simulink model "ROM_draft2"  (R2023a)
settings: Solver=ode15s  StartTime=0.0  StopTime=3  FixedStep=0.1  RelTol=1e-3
model workspace (MAT data in the model file):
  E_IVD4_N = 5
  E_IVD4_Z1 = 5
  E_IVD4_Z2 = 5
  E_IVD4_Z3 = 5
  E_IVD4_Z4 = 5
  E_IVD5_N = 5
  E_IVD5_Z1 = 5
  E_IVD5_Z2 = 5
  E_IVD5_Z3 = 5
  E_IVD5_Z4 = 5
  IVD5_N.InterfaceFrameOrigins = [0.00119634453319  0.0658349886468  0.905560470856; 0.000738781111538  0.0718151805359  0.915203379453]
  IVD5_N.InterfaceFrameOrientations = [0.963982062514  -0.265850048581  -0.0076111073418  0.00209901546435; 0.970389572461  -0.241521069818  0.00331223233616  -0.000824384267944]
  IVD5_N.StiffnessMatrix = [12072.1210467 -274.061579069 -476.370544654 -0.0848536559846 34.5351827952 -19.5673133357 -12072.1210467 274.061579068 476.370544653 -0.121182854467 81.6572072926 -52.5008864779 ... (196 elements, 14x14)]
  IVD5_N.MassMatrix = [0.00145261006911 -3.28751977521e-05 -5.02520057009e-05 2.70896299944e-09 3.95047279511e-07 -1.70980551184e-07 0.000938457476927 1.77908731253e-05 3.15075839837e-05 -9.24765904888e-09 -2.48315227579e-06 1.67944140759e-06 ... (196 elements, 14x14)]
  IVD5_N.GraphicVertexCoordinates = [-0.0121724567413 -0.0105574836731 -0.0114222154617 -0.0129605951309 -0.0126794233322 -0.0115785064697 -0.0118535032272 -0.00319156455994 -0.00319188046455 -0.00571438598633 -4.47452294499e-05 0.00311250649847 ... (1698 elements, 566x3)]
  IVD5_N.GraphicFacetVertexIndices = [1 4 5 8 11 14 17 20 23 26 28 31 ... (3384 elements, 1128x3)]
  IVD5_N.GraphicReconstructionMatrix = [0.339186715765 -0.0243256844818 -0.186223853856 0.294199181327 -0.00640190377512 -0.15234196868 0.195526379715 -0.0060796942636 -0.142913155438 0.244126675106 -0.0106723088514 -0.158139775185 ... (23772 elements, 1698x14)]
  IVD5_Z1.InterfaceFrameOrigins = [0.000873550632761  0.0769295550328  0.898954504373; 0.00103448042212  0.0848390231016  0.908281981027]
  IVD5_Z1.InterfaceFrameOrientations = [0.963982062514  -0.265850048581  -0.0076111073418  0.00209901546435; 0.970389572461  -0.241521069818  0.00331223233616  -0.000824384267944]
  IVD5_Z1.StiffnessMatrix = [5996.43220354 4.30460635168 53.0071518463 0.68427648579 19.4752112689 -31.152810894 -5996.43220354 -4.3046063519 -53.0071518468 -0.305169226095 36.4478396857 -16.2750854071 ... (196 elements, 14x14)]
  IVD5_Z1.MassMatrix = [0.00101136411122 -1.06281560629e-05 -1.3336781227e-05 -3.7152952177e-08 9.78126965242e-08 -1.12543471379e-06 0.00055045795202 6.98371650339e-06 1.00424226413e-05 1.09339655695e-08 -1.9997764811e-06 4.03451089866e-07 ... (196 elements, 14x14)]
  IVD5_Z1.GraphicVertexCoordinates = [-0.00849552154541 -0.00710174512863 -0.00716232396796 -0.0142471482979 -0.0153294525146 -0.0152496709824 -0.00567360639572 -0.00564802122116 -0.00557869402219 -0.00564833688736 -0.00567392206192 0.00247848033905 ... (1554 elements, 518x3)]
  IVD5_Z1.GraphicFacetVertexIndices = [1 4 7 10 10 12 15 18 20 23 26 29 ... (3096 elements, 1032x3)]
  IVD5_Z1.GraphicReconstructionMatrix = [0.199445115194 -0.0696803209522 -0.0744700855901 0.0059035639951 -0.000379739053346 -0.0013061688012 0.0307297998401 -0.0137062851462 -0.0106957383637 0.40254283486 -0.169685115848 -0.185804981554 ... (21756 elements, 1554x14)]
  IVD5_Z2.InterfaceFrameOrigins = [0.000604761990392  0.0571888576031  0.910711195808; 4.49988118865e-05  0.0600241328211  0.921467825643]
  IVD5_Z2.InterfaceFrameOrientations = [0.963982062514  -0.265850048581  -0.0076111073418  0.00209901546435; 0.970389572461  -0.241521069818  0.00331223233616  -0.000824384267944]
  IVD5_Z2.StiffnessMatrix = [3182.87404983 7.23028304405 -81.8198650663 -0.0684213777452 14.0226472063 0.101851145356 -3182.87404983 -7.23028304422 81.8198650673 -0.241333936335 20.1685510133 -9.13022230709 ... (196 elements, 14x14)]
  IVD5_Z2.MassMatrix = [0.000320666483951 4.44068362481e-07 -1.92499536011e-07 -4.69532859899e-09 2.63976402041e-07 3.85211947716e-08 0.000231555416641 1.63281867833e-06 7.22837907777e-07 7.7167688392e-09 -8.23428240926e-07 4.59263039163e-07 ... (196 elements, 14x14)]
  IVD5_Z2.GraphicVertexCoordinates = [0.0116057628963 0.0122282781601 0.0116208400726 -0.0131143016815 -0.0129614706039 -0.0126898040771 -0.0121298876402 -0.0133299627304 -0.0129422960281 -0.0121591796875 -0.0137408895493 -0.0137489080429 ... (1266 elements, 422x3)]
  IVD5_Z2.GraphicFacetVertexIndices = [1 4 4 4 4 9 12 14 17 20 23 25 ... (2520 elements, 840x3)]
  IVD5_Z2.GraphicReconstructionMatrix = [0.022905241299 -0.0160356716758 0.0172326687077 0.174782421627 -0.0165100138029 0.159517344737 0.0018288444813 -0.00446676244893 0.00273822898953 0.452008736901 0.0398453014282 -0.281808352519 ... (17724 elements, 1266x14)]
  IVD5_Z3.InterfaceFrameOrigins = [-0.0141350531982  0.0665747464449  0.90484779108; -0.0154737618286  0.0716573347521  0.915406801231]
  IVD5_Z3.InterfaceFrameOrientations = [0.963982062514  -0.265850048581  -0.0076111073418  0.00209901546435; 0.970389572461  -0.241521069818  0.00331223233616  -0.000824384267944]
  IVD5_Z3.StiffnessMatrix = [4692.3946555 -372.737703142 -764.852122067 4.59128038682 24.6626166315 -13.5635629732 -4692.3946555 372.737703142 764.852122068 -4.54296764783 23.8605120342 -9.7869600556 ... (196 elements, 14x14)]
  IVD5_Z3.MassMatrix = [0.00108979588426 -7.91948772423e-05 -0.00012971252151 -3.95532003515e-07 6.16575573035e-07 -1.62927188642e-06 0.000430209135056 4.56023636695e-05 7.63206897759e-05 3.12965499465e-07 -1.54222628864e-06 5.60394961299e-08 ... (196 elements, 14x14)]
  IVD5_Z3.GraphicVertexCoordinates = [-0.0119716072083 -0.0115785064697 -0.010625453949 -0.0105742545404 -0.00962718868256 -0.0102103004456 -0.00961538410187 -0.00823415184021 -0.00846083084375 -0.00981032980596 -0.0216970863342 -0.0212184925079 ... (1647 elements, 549x3)]
  IVD5_Z3.GraphicFacetVertexIndices = [1 4 7 5 11 11 16 19 22 25 28 28 ... (3282 elements, 1094x3)]
  IVD5_Z3.GraphicReconstructionMatrix = [0.840714753705 0.0133701682388 0.0301596742866 0.935799594756 0.00827310844295 -0.000351030592675 0.928574226604 0.0130189350162 -0.00421675452139 1 0 0 ... (23058 elements, 1647x14)]
  IVD5_Z4.InterfaceFrameOrigins = [0.0154934204985  0.0666268291128  0.905355941171; 0.016602773215  0.0722511228627  0.914848619757]
  IVD5_Z4.InterfaceFrameOrientations = [0.963982062514  -0.265850048581  -0.0076111073418  0.00209901546435; 0.970389572461  -0.241521069818  0.00331223233616  -0.000824384267944]
  IVD5_Z4.StiffnessMatrix = [4497.70767679 485.699170129 728.111952949 -0.284496397968 21.0935467669 -12.2902479984 -4497.7076768 -485.699170128 -728.111952948 -0.230974207325 20.7940136099 -12.4673694835 ... (196 elements, 14x14)]
  IVD5_Z4.MassMatrix = [0.00093076023563 8.043991063e-05 0.000134475236068 1.54197560363e-07 6.30928617545e-07 -7.91605463934e-07 0.00039447557349 -3.908143269e-05 -6.99652139148e-05 -4.27032038908e-08 -1.12100834172e-06 3.82435240934e-07 ... (196 elements, 14x14)]
  IVD5_Z4.GraphicVertexCoordinates = [0.0159857854843 0.0158102636337 0.0160290205696 0.0113312082291 0.0124453754425 0.0113169021606 0.0136561098099 0.0132201137543 0.0159859218597 0.014517357363 0.0145924978256 0.0145923614502 ... (1701 elements, 567x3)]
  IVD5_Z4.GraphicFacetVertexIndices = [1 4 4 9 9 13 16 9 17 17 17 22 ... (3390 elements, 1130x3)]
  IVD5_Z4.GraphicReconstructionMatrix = [0.00193650063384 0.00161007141247 -0.000693027590546 0.190702289547 0.0501215721414 0.0903320858065 0.024566412091 0.00386906829726 0.0109690471668 0.999511548589 0.000299561896416 -0.000263295731636 ... (23814 elements, 1701x14)]
  Moment_AR = 0
  Moment_FE = 0
  Moment_LB = 0
  ROM_draft1_sdosession : sldodialogs.data.SessionData (value not decoded)
  ROM_draft2_sdosession = sldodialogs.data.SessionData
  ROM_draft2_sdosession.Version = '4.0'
  ROM_draft2_sdosession.Data.ModelName = 'ROM_draft2'
  ROM_draft2_sdosession.Data.ToolType = 'ResponseOptimization'
  ROM_draft2_sdosession.Data.GUIOptions.NoPromptClose = 0
  ROM_draft2_sdosession.Data.Workspace.LocalWorkspace.BlockReq = sldodialogs.databrowser.BlockRequirementData
  ROM_draft2_sdosession.Data.Workspace.LocalWorkspace.BlockReq.Name = 'BlockReq'
  ROM_draft2_sdosession.Data.Workspace.LocalWorkspace.BlockReq.Block = 'ROM_draft2/Check AR angle'
  ROM_draft2_sdosession.Data.Workspace.LocalWorkspace.BlockReq_1 = sldodialogs.databrowser.BlockRequirementData
  ROM_draft2_sdosession.Data.Workspace.LocalWorkspace.BlockReq_1.Name = 'BlockReq_1'
  ROM_draft2_sdosession.Data.Workspace.LocalWorkspace.BlockReq_1.Block = 'ROM_draft2/Check FE angle'
  ROM_draft2_sdosession.Data.Workspace.LocalWorkspace.BlockReq_2 = sldodialogs.databrowser.BlockRequirementData
  ROM_draft2_sdosession.Data.Workspace.LocalWorkspace.BlockReq_2.Name = 'BlockReq_2'
  ROM_draft2_sdosession.Data.Workspace.LocalWorkspace.BlockReq_2.Block = 'ROM_draft2/Check LB angle'
  ROM_draft2_sdosession.Data.Workspace.LocalWorkspace.DesignVars(1) = param.Continuous
  ROM_draft2_sdosession.Data.Workspace.LocalWorkspace.DesignVars(1).Minimum_ = 1
  ROM_draft2_sdosession.Data.Workspace.LocalWorkspace.DesignVars(1).Maximum_ = 15
  ROM_draft2_sdosession.Data.Workspace.LocalWorkspace.DesignVars(1).Size_ = [1 1]
  ROM_draft2_sdosession.Data.Workspace.LocalWorkspace.DesignVars(1).Value_ = 10.1302528055
  ROM_draft2_sdosession.Data.Workspace.LocalWorkspace.DesignVars(1).pID = paramid.Variable
  ROM_draft2_sdosession.Data.Workspace.LocalWorkspace.DesignVars(1).pID.Name = 'E_IVD5_N'
  ROM_draft2_sdosession.Data.Workspace.LocalWorkspace.DesignVars(2) = param.Continuous
  ROM_draft2_sdosession.Data.Workspace.LocalWorkspace.DesignVars(2).Minimum_ = 1
  ROM_draft2_sdosession.Data.Workspace.LocalWorkspace.DesignVars(2).Maximum_ = 15
  ROM_draft2_sdosession.Data.Workspace.LocalWorkspace.DesignVars(2).Size_ = [1 1]
  ROM_draft2_sdosession.Data.Workspace.LocalWorkspace.DesignVars(2).Value_ = 10.1799147777
  ROM_draft2_sdosession.Data.Workspace.LocalWorkspace.DesignVars(2).pID = paramid.Variable
  ROM_draft2_sdosession.Data.Workspace.LocalWorkspace.DesignVars(2).pID.Name = 'E_IVD5_Z1'
  ROM_draft2_sdosession.Data.Workspace.LocalWorkspace.DesignVars(3) = param.Continuous
  ROM_draft2_sdosession.Data.Workspace.LocalWorkspace.DesignVars(3).Minimum_ = 1
  ROM_draft2_sdosession.Data.Workspace.LocalWorkspace.DesignVars(3).Maximum_ = 15
  ROM_draft2_sdosession.Data.Workspace.LocalWorkspace.DesignVars(3).Size_ = [1 1]
  ROM_draft2_sdosession.Data.Workspace.LocalWorkspace.DesignVars(3).Value_ = 10.0818306864
  ROM_draft2_sdosession.Data.Workspace.LocalWorkspace.DesignVars(3).pID = paramid.Variable
  ROM_draft2_sdosession.Data.Workspace.LocalWorkspace.DesignVars(3).pID.Name = 'E_IVD5_Z2'
  ROM_draft2_sdosession.Data.Workspace.LocalWorkspace.DesignVars(4) = param.Continuous
  ROM_draft2_sdosession.Data.Workspace.LocalWorkspace.DesignVars(4).Minimum_ = 1
  ROM_draft2_sdosession.Data.Workspace.LocalWorkspace.DesignVars(4).Maximum_ = 15
  ROM_draft2_sdosession.Data.Workspace.LocalWorkspace.DesignVars(4).Size_ = [1 1]
  ROM_draft2_sdosession.Data.Workspace.LocalWorkspace.DesignVars(4).Value_ = 10.2593862475
  ROM_draft2_sdosession.Data.Workspace.LocalWorkspace.DesignVars(4).pID = paramid.Variable
  ROM_draft2_sdosession.Data.Workspace.LocalWorkspace.DesignVars(4).pID.Name = 'E_IVD5_Z3'
  ROM_draft2_sdosession.Data.Workspace.LocalWorkspace.DesignVars(5) = param.Continuous
  ROM_draft2_sdosession.Data.Workspace.LocalWorkspace.DesignVars(5).Minimum_ = 1
  ROM_draft2_sdosession.Data.Workspace.LocalWorkspace.DesignVars(5).Maximum_ = 15
  ROM_draft2_sdosession.Data.Workspace.LocalWorkspace.DesignVars(5).Size_ = [1 1]
  ROM_draft2_sdosession.Data.Workspace.LocalWorkspace.DesignVars(5).Value_ = 10.2473616739
  ROM_draft2_sdosession.Data.Workspace.LocalWorkspace.DesignVars(5).pID = paramid.Variable
  ROM_draft2_sdosession.Data.Workspace.LocalWorkspace.DesignVars(5).pID.Name = 'E_IVD5_Z4'
  ROM_draft2_sdosession.Data.Workspace.LocalWorkspace.ReqValues(1).Name = 'ROM_draft2/Check AR angle (Upper)'
  ROM_draft2_sdosession.Data.Workspace.LocalWorkspace.ReqValues(1).Type = '<='
  ROM_draft2_sdosession.Data.Workspace.LocalWorkspace.ReqValues(1).Value = 0.0202576901416
  ROM_draft2_sdosession.Data.Workspace.LocalWorkspace.ReqValues(1).DisplayValue = 0.0202576901416
  ROM_draft2_sdosession.Data.Workspace.LocalWorkspace.ReqValues(2).Name = 'ROM_draft2/Check AR angle (Lower)'
  ROM_draft2_sdosession.Data.Workspace.LocalWorkspace.ReqValues(2).Type = '>='
  ROM_draft2_sdosession.Data.Workspace.LocalWorkspace.ReqValues(2).Value = -0.00862057830023
  ROM_draft2_sdosession.Data.Workspace.LocalWorkspace.ReqValues(2).DisplayValue = 0.00862057830023
  ROM_draft2_sdosession.Data.Workspace.LocalWorkspace.ReqValues(3).Name = 'ROM_draft2/Check FE angle (Upper)'
  ROM_draft2_sdosession.Data.Workspace.LocalWorkspace.ReqValues(3).Type = '<='
  ROM_draft2_sdosession.Data.Workspace.LocalWorkspace.ReqValues(3).Value = -0.18884415863
  ROM_draft2_sdosession.Data.Workspace.LocalWorkspace.ReqValues(3).DisplayValue = -0.18884415863
  ROM_draft2_sdosession.Data.Workspace.LocalWorkspace.ReqValues(4).Name = 'ROM_draft2/Check FE angle (Lower)'
  ROM_draft2_sdosession.Data.Workspace.LocalWorkspace.ReqValues(4).Type = '>='
  ROM_draft2_sdosession.Data.Workspace.LocalWorkspace.ReqValues(4).Value = -0.186140172919
  ROM_draft2_sdosession.Data.Workspace.LocalWorkspace.ReqValues(4).DisplayValue = 0.186140172919
  ROM_draft2_sdosession.Data.Workspace.LocalWorkspace.ReqValues(5).Name = 'ROM_draft2/Check LB angle (Upper)'
  ROM_draft2_sdosession.Data.Workspace.LocalWorkspace.ReqValues(5).Type = '<='
  ROM_draft2_sdosession.Data.Workspace.LocalWorkspace.ReqValues(5).Value = -0.357049880162
  ROM_draft2_sdosession.Data.Workspace.LocalWorkspace.ReqValues(5).DisplayValue = -0.357049880162
  ROM_draft2_sdosession.Data.Workspace.LocalWorkspace.ReqValues(6).Name = 'ROM_draft2/Check LB angle (Lower)'
  ROM_draft2_sdosession.Data.Workspace.LocalWorkspace.ReqValues(6).Type = '>='
  ROM_draft2_sdosession.Data.Workspace.LocalWorkspace.ReqValues(6).Value = -0.338560110282
  ROM_draft2_sdosession.Data.Workspace.LocalWorkspace.ReqValues(6).DisplayValue = 0.338560110282
  ROM_draft2_sdosession.Data.Workspace.LocalWorkspace.ReqValues_1(1).Name = 'ROM_draft2/Check AR angle (Upper)'
  ROM_draft2_sdosession.Data.Workspace.LocalWorkspace.ReqValues_1(1).Type = '<='
  ROM_draft2_sdosession.Data.Workspace.LocalWorkspace.ReqValues_1(1).Value = -5.6447610177e-05
  ROM_draft2_sdosession.Data.Workspace.LocalWorkspace.ReqValues_1(1).DisplayValue = -5.6447610177e-05
  ROM_draft2_sdosession.Data.Workspace.LocalWorkspace.ReqValues_1(2).Name = 'ROM_draft2/Check AR angle (Lower)'
  ROM_draft2_sdosession.Data.Workspace.LocalWorkspace.ReqValues_1(2).Type = '>='
  ROM_draft2_sdosession.Data.Workspace.LocalWorkspace.ReqValues_1(2).Value = -0.0294000963956
  ROM_draft2_sdosession.Data.Workspace.LocalWorkspace.ReqValues_1(2).DisplayValue = 0.0294000963956
  ROM_draft2_sdosession.Data.Workspace.LocalWorkspace.ReqValues_1(3).Name = 'ROM_draft2/Check FE angle (Upper)'
  ROM_draft2_sdosession.Data.Workspace.LocalWorkspace.ReqValues_1(3).Type = '<='
  ROM_draft2_sdosession.Data.Workspace.LocalWorkspace.ReqValues_1(3).Value = -0.202414273831
  ROM_draft2_sdosession.Data.Workspace.LocalWorkspace.ReqValues_1(3).DisplayValue = -0.202414273831
  ROM_draft2_sdosession.Data.Workspace.LocalWorkspace.ReqValues_1(4).Name = 'ROM_draft2/Check FE angle (Lower)'
  ROM_draft2_sdosession.Data.Workspace.LocalWorkspace.ReqValues_1(4).Type = '>='
  ROM_draft2_sdosession.Data.Workspace.LocalWorkspace.ReqValues_1(4).Value = -0.19968402687
  ROM_draft2_sdosession.Data.Workspace.LocalWorkspace.ReqValues_1(4).DisplayValue = 0.19968402687
  ROM_draft2_sdosession.Data.Workspace.LocalWorkspace.ReqValues_1(5).Name = 'ROM_draft2/Check LB angle (Upper)'
  ROM_draft2_sdosession.Data.Workspace.LocalWorkspace.ReqValues_1(5).Type = '<='
  ROM_draft2_sdosession.Data.Workspace.LocalWorkspace.ReqValues_1(5).Value = -0.37091083584
  ROM_draft2_sdosession.Data.Workspace.LocalWorkspace.ReqValues_1(5).DisplayValue = -0.37091083584
  ROM_draft2_sdosession.Data.Workspace.LocalWorkspace.ReqValues_1(6).Name = 'ROM_draft2/Check LB angle (Lower)'
  ROM_draft2_sdosession.Data.Workspace.LocalWorkspace.ReqValues_1(6).Type = '>='
  ROM_draft2_sdosession.Data.Workspace.LocalWorkspace.ReqValues_1(6).Value = -0.352531979443
  ROM_draft2_sdosession.Data.Workspace.LocalWorkspace.ReqValues_1(6).DisplayValue = 0.352531979443
  ROM_draft2_sdosession.Data.Workspace.HiddenWorkspace = []
  ROM_draft2_sdosession.Data.ToolData.DialogManager = []
  ROM_draft2_sdosession.Data.ToolData.PlotManager.Plots(1).Class = 'block'
  ROM_draft2_sdosession.Data.ToolData.PlotManager.Plots(1).Sources = {'ROM_draft2/Check AR angle'}
  ROM_draft2_sdosession.Data.ToolData.PlotManager.Plots(2).Class = 'block'
  ROM_draft2_sdosession.Data.ToolData.PlotManager.Plots(2).Sources = {'ROM_draft2/Check FE angle'}
  ROM_draft2_sdosession.Data.ToolData.PlotManager.Plots(3).Class = 'block'
  ROM_draft2_sdosession.Data.ToolData.PlotManager.Plots(3).Sources = {'ROM_draft2/Check LB angle'}
  ROM_draft2_sdosession.Data.ToolData.PlotManager.Plots(4).Class = 'sldoplots.IterPlot'
  ROM_draft2_sdosession.Data.ToolData.PlotManager.Plots(4).Sources = {'DesignVars'}
  ROM_draft2_sdosession.Data.ToolData.PlotManager.Tiling.gridDimensions.w = 4
  ROM_draft2_sdosession.Data.ToolData.PlotManager.Tiling.gridDimensions.h = 1
  ROM_draft2_sdosession.Data.ToolData.PlotManager.Tiling.tileCount = 4
  ROM_draft2_sdosession.Data.ToolData.PlotManager.Tiling.tileCoverage = [1 2 3 4]
  ROM_draft2_sdosession.Data.ToolData.PlotManager.Tiling.referenceWidth = 812
  ROM_draft2_sdosession.Data.ToolData.PlotManager.Tiling.referenceHeight = 417
  ROM_draft2_sdosession.Data.ToolData.PlotManager.Tiling.columnWeights = [0.250927070457; 0.249690976514; 0.249690976514; 0.249690976514]
  ROM_draft2_sdosession.Data.ToolData.PlotManager.Tiling.rowWeights = 1
  ROM_draft2_sdosession.Data.ToolData.PlotManager.Tiling.columnLeft = [0; 203; 406; 609; 812]
  ROM_draft2_sdosession.Data.ToolData.PlotManager.Tiling.rowTop = [0; 417]
  ROM_draft2_sdosession.Data.ToolData.PlotManager.Tiling.tileOccupancy(1).children.showOrder = 4
  ROM_draft2_sdosession.Data.ToolData.PlotManager.Tiling.tileOccupancy(1).children.id = 'PlotManager f54af110-036d-408f-8777-6d928fe47f50_TimePlot b304c782-29f9-45ae-8c66-0a2cc5438744'
  ROM_draft2_sdosession.Data.ToolData.PlotManager.Tiling.tileOccupancy(1).children.title = 'Time plot 1'
  ROM_draft2_sdosession.Data.ToolData.PlotManager.Tiling.tileOccupancy(1).showingChildId = 'PlotManager f54af110-036d-408f-8777-6d928fe47f50_TimePlot b304c782-29f9-45ae-8c66-0a2cc5438744'
  ROM_draft2_sdosession.Data.ToolData.PlotManager.Tiling.tileOccupancy(1).showingChildTitle = 'Time plot 1'
  ROM_draft2_sdosession.Data.ToolData.PlotManager.Tiling.tileOccupancy(2).children.showOrder = 0
  ROM_draft2_sdosession.Data.ToolData.PlotManager.Tiling.tileOccupancy(2).children.id = 'PlotManager f54af110-036d-408f-8777-6d928fe47f50_TimePlot dc3739cf-55c9-4e0f-a459-5725c8fe8cac'
  ROM_draft2_sdosession.Data.ToolData.PlotManager.Tiling.tileOccupancy(2).children.title = 'Time plot 3'
  ROM_draft2_sdosession.Data.ToolData.PlotManager.Tiling.tileOccupancy(2).showingChildId = 'PlotManager f54af110-036d-408f-8777-6d928fe47f50_TimePlot dc3739cf-55c9-4e0f-a459-5725c8fe8cac'
  ROM_draft2_sdosession.Data.ToolData.PlotManager.Tiling.tileOccupancy(2).showingChildTitle = 'Time plot 3'
  ROM_draft2_sdosession.Data.ToolData.PlotManager.Tiling.tileOccupancy(3).children.showOrder = 2
  ROM_draft2_sdosession.Data.ToolData.PlotManager.Tiling.tileOccupancy(3).children.id = 'PlotManager f54af110-036d-408f-8777-6d928fe47f50_TimePlot eb6b7a91-08b8-42c7-b08f-fe9f82b9e88b'
  ROM_draft2_sdosession.Data.ToolData.PlotManager.Tiling.tileOccupancy(3).children.title = 'Time plot 2'
  ROM_draft2_sdosession.Data.ToolData.PlotManager.Tiling.tileOccupancy(3).showingChildId = 'PlotManager f54af110-036d-408f-8777-6d928fe47f50_TimePlot eb6b7a91-08b8-42c7-b08f-fe9f82b9e88b'
  ROM_draft2_sdosession.Data.ToolData.PlotManager.Tiling.tileOccupancy(3).showingChildTitle = 'Time plot 2'
  ROM_draft2_sdosession.Data.ToolData.PlotManager.Tiling.tileOccupancy(4).children.showOrder = 0
  ROM_draft2_sdosession.Data.ToolData.PlotManager.Tiling.tileOccupancy(4).children.id = 'PlotManager f54af110-036d-408f-8777-6d928fe47f50_IterPlot fb6630e6-6a22-458a-8f31-b930ee776144'
  ROM_draft2_sdosession.Data.ToolData.PlotManager.Tiling.tileOccupancy(4).children.title = 'DesignVars'
  ROM_draft2_sdosession.Data.ToolData.PlotManager.Tiling.tileOccupancy(4).showingChildId = 'PlotManager f54af110-036d-408f-8777-6d928fe47f50_IterPlot fb6630e6-6a22-458a-8f31-b930ee776144'
  ROM_draft2_sdosession.Data.ToolData.PlotManager.Tiling.tileOccupancy(4).showingChildTitle = 'DesignVars'
  ROM_draft2_sdosession.Data.ToolData.PlotManager.Tiling.emptyTileCount = 0
  ROM_draft2_sdosession.Data.ToolData.PlotManager.Tiling.selectionOrder.PlotManagerF54af110_036d_408f_8777_6d928fe47f50_TimePlotB304c78 = 0
  ROM_draft2_sdosession.Data.ToolData.PlotManager.Tiling.selectionOrder.PlotManagerF54af110_036d_408f_8777_6d928fe47f50_TimePlotDc3739c = 1
  ROM_draft2_sdosession.Data.ToolData.PlotManager.Tiling.selectionOrder.PlotManagerF54af110_036d_408f_8777_6d928fe47f50_TimePlotEb6b7a9 = 5
  ROM_draft2_sdosession.Data.ToolData.PlotManager.Tiling.selectionOrder.PlotManagerF54af110_036d_408f_8777_6d928fe47f50_IterPlotFb6630e = 7
  ROM_draft2_sdosession.Data.ToolData.ResponseOptimization.Options = sdo.OptimizeOptions
  ROM_draft2_sdosession.Data.ToolData.ResponseOptimization.Options.OptimizedModel = 'ROM_draft2'
  ROM_draft2_sdosession.Data.ToolData.ResponseOptimization.Options.Version = 2
  ROM_draft2_sdosession.Data.ToolData.ResponseOptimization.GUIOptions.ModelTimeOut = Inf
  ROM_draft2_sdosession.Data.ToolData.ResponseOptimization.GUIOptions.ComputeOperatingPoint = 0
  ROM_draft2_sdosession.Data.ToolData.ResponseOptimization.GUIOptions.ShowProgress = 1
  ROM_draft2_sdosession.Data.ToolData.ResponseOptimization.GUIOptions.ShowParamTrajectory = 1
  ROM_draft2_sdosession.Data.ToolData.ResponseOptimization.GUIOptions.UpdatePlots = 1
  ROM_draft2_sdosession.Data.ToolData.ResponseOptimization.GUIOptions.UpdateModel = 1
  ROM_draft2_sdosession.Data.ToolData.ResponseOptimization.GUIOptions.UpdateDesign = 'overwrite'
  ROM_draft2_sdosession.Data.ToolData.ResponseOptimization.GUIOptions.SaveReport = 0
  ROM_draft2_sdosession.Data.ToolData.ResponseOptimization.GUIOptions.SaveRequirementValue = 1
  ROM_draft2_sdosession.Data.ToolData.ResponseOptimization.RequirementOperatingPointSetup = []
  ROM_draft2_sdosession.Data.ToolData.ResponseOptimization.LocalRequirements = struct([])
  ROM_draft2_sdosession.Data.ToolData.ResponseOptimization.BlockRequirements(1).Block = 'ROM_draft2/Check AR angle'
  ROM_draft2_sdosession.Data.ToolData.ResponseOptimization.BlockRequirements(1).Selected = 1
  ROM_draft2_sdosession.Data.ToolData.ResponseOptimization.BlockRequirements(1).hReq(1) = sdo.requirements.SignalBound
  ROM_draft2_sdosession.Data.ToolData.ResponseOptimization.BlockRequirements(1).hReq(1).sdo.requirements.Requirement.Data_ : srorequirement.piecewisedata (value not decoded)
  ROM_draft2_sdosession.Data.ToolData.ResponseOptimization.BlockRequirements(1).hReq(1).sdo.requirements.Requirement.Check_ = sdo.requirements.PiecewiseLinearCheck
  ROM_draft2_sdosession.Data.ToolData.ResponseOptimization.BlockRequirements(1).hReq(1).sdo.requirements.Requirement.Check_.Orientation = 'horizontal'
  ROM_draft2_sdosession.Data.ToolData.ResponseOptimization.BlockRequirements(1).hReq(1).sdo.requirements.Requirement.Check_.XScale = 'linear'
  ROM_draft2_sdosession.Data.ToolData.ResponseOptimization.BlockRequirements(1).hReq(2) = sdo.requirements.SignalBound
  ROM_draft2_sdosession.Data.ToolData.ResponseOptimization.BlockRequirements(1).hReq(2).sdo.requirements.Requirement.Data_ : srorequirement.piecewisedata (value not decoded)
  ROM_draft2_sdosession.Data.ToolData.ResponseOptimization.BlockRequirements(1).hReq(2).sdo.requirements.Requirement.Check_ = sdo.requirements.PiecewiseLinearCheck
  ROM_draft2_sdosession.Data.ToolData.ResponseOptimization.BlockRequirements(1).hReq(2).sdo.requirements.Requirement.Check_.Orientation = 'horizontal'
  ROM_draft2_sdosession.Data.ToolData.ResponseOptimization.BlockRequirements(1).hReq(2).sdo.requirements.Requirement.Check_.XScale = 'linear'
  ROM_draft2_sdosession.Data.ToolData.ResponseOptimization.BlockRequirements(2).Block = 'ROM_draft2/Check FE angle'
  ROM_draft2_sdosession.Data.ToolData.ResponseOptimization.BlockRequirements(2).Selected = 1
  ROM_draft2_sdosession.Data.ToolData.ResponseOptimization.BlockRequirements(2).hReq(1) = sdo.requirements.SignalBound
  ROM_draft2_sdosession.Data.ToolData.ResponseOptimization.BlockRequirements(2).hReq(1).sdo.requirements.Requirement.Data_ : srorequirement.piecewisedata (value not decoded)
  ROM_draft2_sdosession.Data.ToolData.ResponseOptimization.BlockRequirements(2).hReq(1).sdo.requirements.Requirement.Check_ = sdo.requirements.PiecewiseLinearCheck
  ROM_draft2_sdosession.Data.ToolData.ResponseOptimization.BlockRequirements(2).hReq(1).sdo.requirements.Requirement.Check_.Orientation = 'horizontal'
  ROM_draft2_sdosession.Data.ToolData.ResponseOptimization.BlockRequirements(2).hReq(1).sdo.requirements.Requirement.Check_.XScale = 'linear'
  ROM_draft2_sdosession.Data.ToolData.ResponseOptimization.BlockRequirements(2).hReq(2) = sdo.requirements.SignalBound
  ROM_draft2_sdosession.Data.ToolData.ResponseOptimization.BlockRequirements(2).hReq(2).sdo.requirements.Requirement.Data_ : srorequirement.piecewisedata (value not decoded)
  ROM_draft2_sdosession.Data.ToolData.ResponseOptimization.BlockRequirements(2).hReq(2).sdo.requirements.Requirement.Check_ = sdo.requirements.PiecewiseLinearCheck
  ROM_draft2_sdosession.Data.ToolData.ResponseOptimization.BlockRequirements(2).hReq(2).sdo.requirements.Requirement.Check_.Orientation = 'horizontal'
  ROM_draft2_sdosession.Data.ToolData.ResponseOptimization.BlockRequirements(2).hReq(2).sdo.requirements.Requirement.Check_.XScale = 'linear'
  ROM_draft2_sdosession.Data.ToolData.ResponseOptimization.BlockRequirements(3).Block = 'ROM_draft2/Check LB angle'
  ROM_draft2_sdosession.Data.ToolData.ResponseOptimization.BlockRequirements(3).Selected = 1
  ROM_draft2_sdosession.Data.ToolData.ResponseOptimization.BlockRequirements(3).hReq(1) = sdo.requirements.SignalBound
  ROM_draft2_sdosession.Data.ToolData.ResponseOptimization.BlockRequirements(3).hReq(1).sdo.requirements.Requirement.Data_ : srorequirement.piecewisedata (value not decoded)
  ROM_draft2_sdosession.Data.ToolData.ResponseOptimization.BlockRequirements(3).hReq(1).sdo.requirements.Requirement.Check_ = sdo.requirements.PiecewiseLinearCheck
  ROM_draft2_sdosession.Data.ToolData.ResponseOptimization.BlockRequirements(3).hReq(1).sdo.requirements.Requirement.Check_.Orientation = 'horizontal'
  ROM_draft2_sdosession.Data.ToolData.ResponseOptimization.BlockRequirements(3).hReq(1).sdo.requirements.Requirement.Check_.XScale = 'linear'
  ROM_draft2_sdosession.Data.ToolData.ResponseOptimization.BlockRequirements(3).hReq(2) = sdo.requirements.SignalBound
  ROM_draft2_sdosession.Data.ToolData.ResponseOptimization.BlockRequirements(3).hReq(2).sdo.requirements.Requirement.Data_ : srorequirement.piecewisedata (value not decoded)
  ROM_draft2_sdosession.Data.ToolData.ResponseOptimization.BlockRequirements(3).hReq(2).sdo.requirements.Requirement.Check_ = sdo.requirements.PiecewiseLinearCheck
  ROM_draft2_sdosession.Data.ToolData.ResponseOptimization.BlockRequirements(3).hReq(2).sdo.requirements.Requirement.Check_.Orientation = 'horizontal'
  ROM_draft2_sdosession.Data.ToolData.ResponseOptimization.BlockRequirements(3).hReq(2).sdo.requirements.Requirement.Check_.XScale = 'linear'
  ROM_draft2_sdosession.Data.ToolData.ResponseOptimization.LocalExperiments = struct([])
  ROM_draft2_sdosession.Data.ToolData.ResponseOptimization.Cost.Type = 'SSE'
  ROM_draft2_sdosession.Data.ToolData.ResponseOptimization.Cost.Robust = 'off'
  ROM_draft2_sdosession.Data.ToolData.ResponseOptimization.DesignVariables = 'DesignVars'
  ROM_draft2_sdosession.Data.ToolData.ResponseOptimization.UncertainVariables = ''
  ROM_draft2_sdosession.Data.ToolData.ResponseOptimization.DataToPlot = 'DesignVars'
undefined symbols (not defined in the file): IVD4_N, IVD4_Z1, IVD4_Z2, IVD4_Z3, IVD4_Z4
libraries: sm_lib x29, nesl_utility x9, checkpacklib x4, simulink_extras x4, simulink x1
(part 1 of 2)
settings Model: Creator=siril  LastModifiedBy=siril

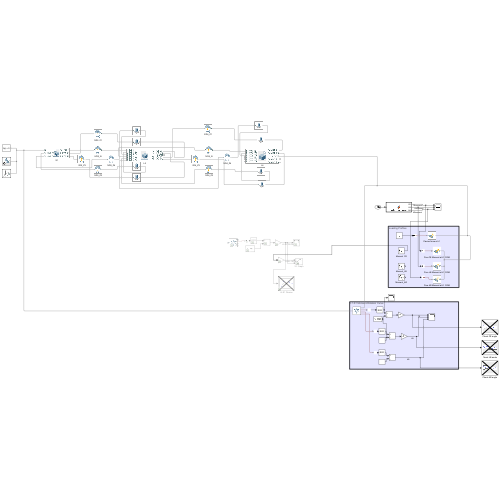
[thumbnail: Simulink's stored preview of the top-level diagram]
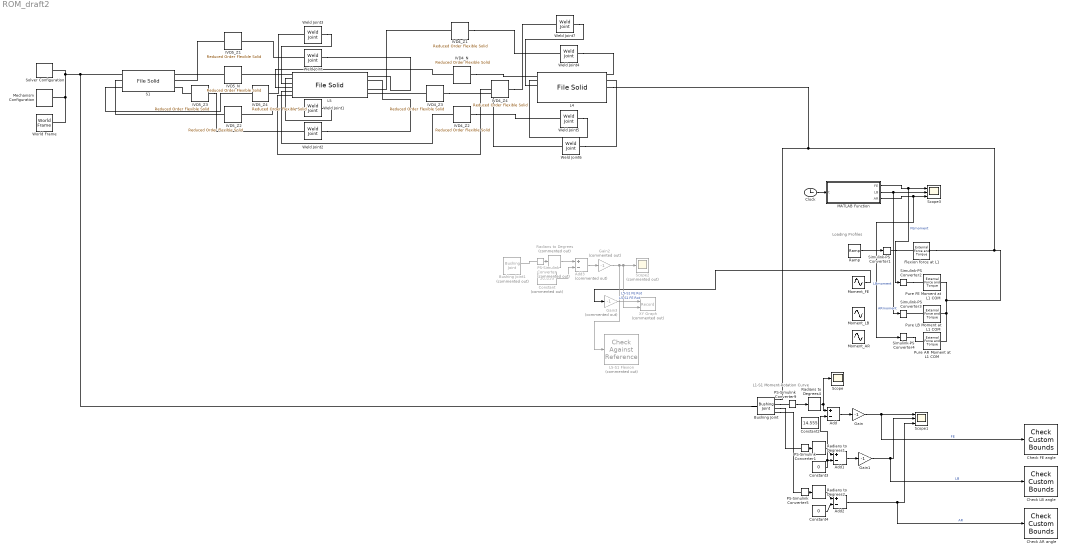
== system ROM_draft2 ==
  note: L1-S1 Moment-Rotation Curve
  note: Loading Profiles
  Add : Sum  Inputs=+-
  Add1 : Sum  Inputs=+-
  Add2 : Sum  Inputs=+-
  Add3 : Sum  Commented=on  Inputs=+-
  Bushing Joint : sm_lib/Joints/Bushing Joint  JointMode=Normal  SenseConstraintForce=off  SenseConstraintForceX=off  SenseConstraintForceY=off  SenseConstraintForceZ=off  SenseConstraintTorque=off  SenseConstraintTorqueX=off  SenseConstraintTorqueY=off  SenseConstraintTorqueZ=off  SenseTotalForce=off  SenseTotalForceX=off  SenseTotalForceY=off  SenseTotalForceZ=off  SenseTotalTorque=off  SenseTotalTorqueX=off  SenseTotalTorqueY=off  SenseTotalTorqueZ=off  CompositeWrenchDir=FollowerOnBase  CompositeWrenchFrame=BaseFrame  PxEquilibriumPosition=0  PxEquilibriumPositionUnits=m  PxSpringStiffness=0  PxSpringStiffnessUnits=N/m  PxDampingCoefficient=0  PxDampingCoefficientUnits=N/(m/s)  PxTorqueActuationMode=NoTorque  PxMotionActuationMode=ComputedMotion  PxSensePosition=off  PxSenseVelocity=off  PxSenseAcceleration=off  PxSenseTorqueForce=off  PxSenseLowerLimitTorqueForce=off  PxSenseUpperLimitTorqueForce=off  PxLowerLimitSpecify=off  PxLowerLimitBound=-1  PxLowerLimitBoundUnits=m  PxLowerLimitStiffness=1e6  PxLowerLimitStiffnessUnits=N/m  PxLowerLimitDamping=1e3  PxLowerLimitDampingUnits=N/(m/s)  PxLowerLimitTransitionRegionWidth=1e-4  PxLowerLimitTransitionRegionWidthUnits=m  PxUpperLimitSpecify=off  PxUpperLimitBound=1  PxUpperLimitBoundUnits=m  PxUpperLimitStiffness=1e6  PxUpperLimitStiffnessUnits=N/m  PxUpperLimitDamping=1e3  PxUpperLimitDampingUnits=N/(m/s)  PxUpperLimitTransitionRegionWidth=1e-4  PxUpperLimitTransitionRegionWidthUnits=m  PxPositionTargetSpecify=off  PxPositionTargetPriority=High  PxPositionTargetValue=0  PxPositionTargetValueUnits=m  PxVelocityTargetSpecify=off  PxVelocityTargetPriority=High  PxVelocityTargetValue=0  PxVelocityTargetValueUnits=m/s  PyEquilibriumPosition=0  PyEquilibriumPositionUnits=m  PySpringStiffness=0  PySpringStiffnessUnits=N/m  PyDampingCoefficient=0  PyDampingCoefficientUnits=N/(m/s)  PyTorqueActuationMode=NoTorque  PyMotionActuationMode=ComputedMotion  PySensePosition=off  PySenseVelocity=off  PySenseAcceleration=off  PySenseTorqueForce=off  PySenseLowerLimitTorqueForce=off  PySenseUpperLimitTorqueForce=off  PyLowerLimitSpecify=off  PyLowerLimitBound=-1  PyLowerLimitBoundUnits=m  PyLowerLimitStiffness=1e6  PyLowerLimitStiffnessUnits=N/m  PyLowerLimitDamping=1e3  PyLowerLimitDampingUnits=N/(m/s)  PyLowerLimitTransitionRegionWidth=1e-4  PyLowerLimitTransitionRegionWidthUnits=m  PyUpperLimitSpecify=off  PyUpperLimitBound=1  PyUpperLimitBoundUnits=m  PyUpperLimitStiffness=1e6  PyUpperLimitStiffnessUnits=N/m  PyUpperLimitDamping=1e3  PyUpperLimitDampingUnits=N/(m/s)  PyUpperLimitTransitionRegionWidth=1e-4  PyUpperLimitTransitionRegionWidthUnits=m  PyPositionTargetSpecify=off  PyPositionTargetPriority=High  PyPositionTargetValue=0  PyPositionTargetValueUnits=m  PyVelocityTargetSpecify=off  PyVelocityTargetPriority=High  PyVelocityTargetValue=0  PyVelocityTargetValueUnits=m/s  PzEquilibriumPosition=0  PzEquilibriumPositionUnits=m  PzSpringStiffness=0  PzSpringStiffnessUnits=N/m  PzDampingCoefficient=0  PzDampingCoefficientUnits=N/(m/s)  PzTorqueActuationMode=NoTorque  PzMotionActuationMode=ComputedMotion  PzSensePosition=off  PzSenseVelocity=off  PzSenseAcceleration=off  PzSenseTorqueForce=off  PzSenseLowerLimitTorqueForce=off  PzSenseUpperLimitTorqueForce=off  PzLowerLimitSpecify=off  PzLowerLimitBound=-1  PzLowerLimitBoundUnits=m  PzLowerLimitStiffness=1e6  PzLowerLimitStiffnessUnits=N/m  PzLowerLimitDamping=1e3  PzLowerLimitDampingUnits=N/(m/s)  PzLowerLimitTransitionRegionWidth=1e-4  PzLowerLimitTransitionRegionWidthUnits=m  PzUpperLimitSpecify=off  PzUpperLimitBound=1  PzUpperLimitBoundUnits=m  PzUpperLimitStiffness=1e6  PzUpperLimitStiffnessUnits=N/m  PzUpperLimitDamping=1e3  PzUpperLimitDampingUnits=N/(m/s)  PzUpperLimitTransitionRegionWidth=1e-4  PzUpperLimitTransitionRegionWidthUnits=m  PzPositionTargetSpecify=off  PzPositionTargetPriority=High  PzPositionTargetValue=0  PzPositionTargetValueUnits=m  PzVelocityTargetSpecify=off  PzVelocityTargetPriority=High  PzVelocityTargetValue=0  PzVelocityTargetValueUnits=m/s  RxEquilibriumPosition=0  RxEquilibriumPositionUnits=deg  RxSpringStiffness=0  RxSpringStiffnessUnits=N*m/deg  RxDampingCoefficient=0  RxDampingCoefficientUnits=N*m/(deg/s)  RxTorqueActuationMode=NoTorque  RxMotionActuationMode=ComputedMotion  RxSensePosition=on  RxSenseVelocity=off  RxSenseAcceleration=off  RxSenseTorqueForce=off  RxSenseLowerLimitTorqueForce=off  RxSenseUpperLimitTorqueForce=off  RxLowerLimitSpecify=off  RxLowerLimitBound=-90  RxLowerLimitBoundUnits=deg  RxLowerLimitStiffness=1e4  RxLowerLimitStiffnessUnits=N*m/deg  RxLowerLimitDamping=10  RxLowerLimitDampingUnits=N*m/(deg/s)  RxLowerLimitTransitionRegionWidth=0.1  RxLowerLimitTransitionRegionWidthUnits=deg  RxUpperLimitSpecify=off  RxUpperLimitBound=90  RxUpperLimitBoundUnits=deg  RxUpperLimitStiffness=1e4  RxUpperLimitStiffnessUnits=N*m/deg  RxUpperLimitDamping=10  RxUpperLimitDampingUnits=N*m/(deg/s)  RxUpperLimitTransitionRegionWidth=0.1  RxUpperLimitTransitionRegionWidthUnits=deg  RxPositionTargetSpecify=off  RxPositionTargetPriority=High  RxPositionTargetValue=0  RxPositionTargetValueUnits=deg  RxVelocityTargetSpecify=off  RxVelocityTargetPriority=High  RxVelocityTargetValue=0  RxVelocityTargetValueUnits=deg/s  RyEquilibriumPosition=0  RyEquilibriumPositionUnits=deg  RySpringStiffness=0  RySpringStiffnessUnits=N*m/deg  RyDampingCoefficient=0  RyDampingCoefficientUnits=N*m/(deg/s)  RyTorqueActuationMode=NoTorque  RyMotionActuationMode=ComputedMotion  RySensePosition=on  RySenseVelocity=off  RySenseAcceleration=off  RySenseTorqueForce=off  RySenseLowerLimitTorqueForce=off  RySenseUpperLimitTorqueForce=off  RyLowerLimitSpecify=off  RyLowerLimitBound=-90  RyLowerLimitBoundUnits=deg  RyLowerLimitStiffness=1e4  RyLowerLimitStiffnessUnits=N*m/deg  RyLowerLimitDamping=10  RyLowerLimitDampingUnits=N*m/(deg/s)  RyLowerLimitTransitionRegionWidth=0.1  RyLowerLimitTransitionRegionWidthUnits=deg  RyUpperLimitSpecify=off  RyUpperLimitBound=90  RyUpperLimitBoundUnits=deg  RyUpperLimitStiffness=1e4  RyUpperLimitStiffnessUnits=N*m/deg  RyUpperLimitDamping=10  RyUpperLimitDampingUnits=N*m/(deg/s)  RyUpperLimitTransitionRegionWidth=0.1  RyUpperLimitTransitionRegionWidthUnits=deg  RyPositionTargetSpecify=off  RyPositionTargetPriority=High  RyPositionTargetValue=0  RyPositionTargetValueUnits=deg  RyVelocityTargetSpecify=off  RyVelocityTargetPriority=High  RyVelocityTargetValue=0  RyVelocityTargetValueUnits=deg/s  RzEquilibriumPosition=0  RzEquilibriumPositionUnits=deg  RzSpringStiffness=0  RzSpringStiffnessUnits=N*m/deg  RzDampingCoefficient=0  RzDampingCoefficientUnits=N*m/(deg/s)  RzTorqueActuationMode=NoTorque  RzMotionActuationMode=ComputedMotion  RzSensePosition=on  RzSenseVelocity=off  RzSenseAcceleration=off  RzSenseTorqueForce=off  RzSenseLowerLimitTorqueForce=off  RzSenseUpperLimitTorqueForce=off  RzLowerLimitSpecify=off  RzLowerLimitBound=-90  RzLowerLimitBoundUnits=deg  RzLowerLimitStiffness=1e4  RzLowerLimitStiffnessUnits=N*m/deg  RzLowerLimitDamping=10  RzLowerLimitDampingUnits=N*m/(deg/s)  RzLowerLimitTransitionRegionWidth=0.1  RzLowerLimitTransitionRegionWidthUnits=deg  RzUpperLimitSpecify=off  RzUpperLimitBound=90  RzUpperLimitBoundUnits=deg  RzUpperLimitStiffness=1e4  RzUpperLimitStiffnessUnits=N*m/deg  RzUpperLimitDamping=10  RzUpperLimitDampingUnits=N*m/(deg/s)  RzUpperLimitTransitionRegionWidth=0.1  RzUpperLimitTransitionRegionWidthUnits=deg  RzPositionTargetSpecify=off  RzPositionTargetPriority=High  RzPositionTargetValue=0  RzPositionTargetValueUnits=deg  RzVelocityTargetSpecify=off  RzVelocityTargetPriority=High  RzVelocityTargetValue=0  RzVelocityTargetValueUnits=deg/s
  Bushing Joint1 : sm_lib/Joints/Bushing Joint  Commented=on  JointMode=Normal  SenseConstraintForce=off  SenseConstraintForceX=off  SenseConstraintForceY=off  SenseConstraintForceZ=off  SenseConstraintTorque=off  SenseConstraintTorqueX=off  SenseConstraintTorqueY=off  SenseConstraintTorqueZ=off  SenseTotalForce=off  SenseTotalForceX=off  SenseTotalForceY=off  SenseTotalForceZ=off  SenseTotalTorque=off  SenseTotalTorqueX=off  SenseTotalTorqueY=off  SenseTotalTorqueZ=off  CompositeWrenchDir=FollowerOnBase  CompositeWrenchFrame=BaseFrame  PxEquilibriumPosition=0  PxEquilibriumPositionUnits=m  PxSpringStiffness=0  PxSpringStiffnessUnits=N/m  PxDampingCoefficient=0  PxDampingCoefficientUnits=N/(m/s)  PxTorqueActuationMode=NoTorque  PxMotionActuationMode=ComputedMotion  PxSensePosition=off  PxSenseVelocity=off  PxSenseAcceleration=off  PxSenseTorqueForce=off  PxSenseLowerLimitTorqueForce=off  PxSenseUpperLimitTorqueForce=off  PxLowerLimitSpecify=off  PxLowerLimitBound=-1  PxLowerLimitBoundUnits=m  PxLowerLimitStiffness=1e6  PxLowerLimitStiffnessUnits=N/m  PxLowerLimitDamping=1e3  PxLowerLimitDampingUnits=N/(m/s)  PxLowerLimitTransitionRegionWidth=1e-4  PxLowerLimitTransitionRegionWidthUnits=m  PxUpperLimitSpecify=off  PxUpperLimitBound=1  PxUpperLimitBoundUnits=m  PxUpperLimitStiffness=1e6  PxUpperLimitStiffnessUnits=N/m  PxUpperLimitDamping=1e3  PxUpperLimitDampingUnits=N/(m/s)  PxUpperLimitTransitionRegionWidth=1e-4  PxUpperLimitTransitionRegionWidthUnits=m  PxPositionTargetSpecify=off  PxPositionTargetPriority=High  PxPositionTargetValue=0  PxPositionTargetValueUnits=m  PxVelocityTargetSpecify=off  PxVelocityTargetPriority=High  PxVelocityTargetValue=0  PxVelocityTargetValueUnits=m/s  PyEquilibriumPosition=0  PyEquilibriumPositionUnits=m  PySpringStiffness=0  PySpringStiffnessUnits=N/m  PyDampingCoefficient=0  PyDampingCoefficientUnits=N/(m/s)  PyTorqueActuationMode=NoTorque  PyMotionActuationMode=ComputedMotion  PySensePosition=off  PySenseVelocity=off  PySenseAcceleration=off  PySenseTorqueForce=off  PySenseLowerLimitTorqueForce=off  PySenseUpperLimitTorqueForce=off  PyLowerLimitSpecify=off  PyLowerLimitBound=-1  PyLowerLimitBoundUnits=m  PyLowerLimitStiffness=1e6  PyLowerLimitStiffnessUnits=N/m  PyLowerLimitDamping=1e3  PyLowerLimitDampingUnits=N/(m/s)  PyLowerLimitTransitionRegionWidth=1e-4  PyLowerLimitTransitionRegionWidthUnits=m  PyUpperLimitSpecify=off  PyUpperLimitBound=1  PyUpperLimitBoundUnits=m  PyUpperLimitStiffness=1e6  PyUpperLimitStiffnessUnits=N/m  PyUpperLimitDamping=1e3  PyUpperLimitDampingUnits=N/(m/s)  PyUpperLimitTransitionRegionWidth=1e-4  PyUpperLimitTransitionRegionWidthUnits=m  PyPositionTargetSpecify=off  PyPositionTargetPriority=High  PyPositionTargetValue=0  PyPositionTargetValueUnits=m  PyVelocityTargetSpecify=off  PyVelocityTargetPriority=High  PyVelocityTargetValue=0  PyVelocityTargetValueUnits=m/s  PzEquilibriumPosition=0  PzEquilibriumPositionUnits=m  PzSpringStiffness=0  PzSpringStiffnessUnits=N/m  PzDampingCoefficient=0  PzDampingCoefficientUnits=N/(m/s)  PzTorqueActuationMode=NoTorque  PzMotionActuationMode=ComputedMotion  PzSensePosition=off  PzSenseVelocity=off  PzSenseAcceleration=off  PzSenseTorqueForce=off  PzSenseLowerLimitTorqueForce=off  PzSenseUpperLimitTorqueForce=off  PzLowerLimitSpecify=off  PzLowerLimitBound=-1  PzLowerLimitBoundUnits=m  PzLowerLimitStiffness=1e6  PzLowerLimitStiffnessUnits=N/m  PzLowerLimitDamping=1e3  PzLowerLimitDampingUnits=N/(m/s)  PzLowerLimitTransitionRegionWidth=1e-4  PzLowerLimitTransitionRegionWidthUnits=m  PzUpperLimitSpecify=off  PzUpperLimitBound=1  PzUpperLimitBoundUnits=m  PzUpperLimitStiffness=1e6  PzUpperLimitStiffnessUnits=N/m  PzUpperLimitDamping=1e3  PzUpperLimitDampingUnits=N/(m/s)  PzUpperLimitTransitionRegionWidth=1e-4  PzUpperLimitTransitionRegionWidthUnits=m  PzPositionTargetSpecify=off  PzPositionTargetPriority=High  PzPositionTargetValue=0  PzPositionTargetValueUnits=m  PzVelocityTargetSpecify=off  PzVelocityTargetPriority=High  PzVelocityTargetValue=0  PzVelocityTargetValueUnits=m/s  RxEquilibriumPosition=0  RxEquilibriumPositionUnits=deg  RxSpringStiffness=0  RxSpringStiffnessUnits=N*m/deg  RxDampingCoefficient=0  RxDampingCoefficientUnits=N*m/(deg/s)  RxTorqueActuationMode=NoTorque  RxMotionActuationMode=ComputedMotion  RxSensePosition=on  RxSenseVelocity=off  RxSenseAcceleration=off  RxSenseTorqueForce=off  RxSenseLowerLimitTorqueForce=off  RxSenseUpperLimitTorqueForce=off  RxLowerLimitSpecify=off  RxLowerLimitBound=-90  RxLowerLimitBoundUnits=deg  RxLowerLimitStiffness=1e4  RxLowerLimitStiffnessUnits=N*m/deg  RxLowerLimitDamping=10  RxLowerLimitDampingUnits=N*m/(deg/s)  RxLowerLimitTransitionRegionWidth=0.1  RxLowerLimitTransitionRegionWidthUnits=deg  RxUpperLimitSpecify=off  RxUpperLimitBound=90  RxUpperLimitBoundUnits=deg  RxUpperLimitStiffness=1e4  RxUpperLimitStiffnessUnits=N*m/deg  RxUpperLimitDamping=10  RxUpperLimitDampingUnits=N*m/(deg/s)  RxUpperLimitTransitionRegionWidth=0.1  RxUpperLimitTransitionRegionWidthUnits=deg  RxPositionTargetSpecify=off  RxPositionTargetPriority=High  RxPositionTargetValue=0  RxPositionTargetValueUnits=deg  RxVelocityTargetSpecify=off  RxVelocityTargetPriority=High  RxVelocityTargetValue=0  RxVelocityTargetValueUnits=deg/s  RyEquilibriumPosition=0  RyEquilibriumPositionUnits=deg  RySpringStiffness=0  RySpringStiffnessUnits=N*m/deg  RyDampingCoefficient=0  RyDampingCoefficientUnits=N*m/(deg/s)  RyTorqueActuationMode=NoTorque  RyMotionActuationMode=ComputedMotion  RySensePosition=on  RySenseVelocity=off  RySenseAcceleration=off  RySenseTorqueForce=off  RySenseLowerLimitTorqueForce=off  RySenseUpperLimitTorqueForce=off  RyLowerLimitSpecify=off  RyLowerLimitBound=-90  RyLowerLimitBoundUnits=deg  RyLowerLimitStiffness=1e4  RyLowerLimitStiffnessUnits=N*m/deg  RyLowerLimitDamping=10  RyLowerLimitDampingUnits=N*m/(deg/s)  RyLowerLimitTransitionRegionWidth=0.1  RyLowerLimitTransitionRegionWidthUnits=deg  RyUpperLimitSpecify=off  RyUpperLimitBound=90  RyUpperLimitBoundUnits=deg  RyUpperLimitStiffness=1e4  RyUpperLimitStiffnessUnits=N*m/deg  RyUpperLimitDamping=10  RyUpperLimitDampingUnits=N*m/(deg/s)  RyUpperLimitTransitionRegionWidth=0.1  RyUpperLimitTransitionRegionWidthUnits=deg  RyPositionTargetSpecify=off  RyPositionTargetPriority=High  RyPositionTargetValue=0  RyPositionTargetValueUnits=deg  RyVelocityTargetSpecify=off  RyVelocityTargetPriority=High  RyVelocityTargetValue=0  RyVelocityTargetValueUnits=deg/s  RzEquilibriumPosition=0  RzEquilibriumPositionUnits=deg  RzSpringStiffness=0  RzSpringStiffnessUnits=N*m/deg  RzDampingCoefficient=0  RzDampingCoefficientUnits=N*m/(deg/s)  RzTorqueActuationMode=NoTorque  RzMotionActuationMode=ComputedMotion  RzSensePosition=on  RzSenseVelocity=off  RzSenseAcceleration=off  RzSenseTorqueForce=off  RzSenseLowerLimitTorqueForce=off  RzSenseUpperLimitTorqueForce=off  RzLowerLimitSpecify=off  RzLowerLimitBound=-90  RzLowerLimitBoundUnits=deg  RzLowerLimitStiffness=1e4  RzLowerLimitStiffnessUnits=N*m/deg  RzLowerLimitDamping=10  RzLowerLimitDampingUnits=N*m/(deg/s)  RzLowerLimitTransitionRegionWidth=0.1  RzLowerLimitTransitionRegionWidthUnits=deg  RzUpperLimitSpecify=off  RzUpperLimitBound=90  RzUpperLimitBoundUnits=deg  RzUpperLimitStiffness=1e4  RzUpperLimitStiffnessUnits=N*m/deg  RzUpperLimitDamping=10  RzUpperLimitDampingUnits=N*m/(deg/s)  RzUpperLimitTransitionRegionWidth=0.1  RzUpperLimitTransitionRegionWidthUnits=deg  RzPositionTargetSpecify=off  RzPositionTargetPriority=High  RzPositionTargetValue=0  RzPositionTargetValueUnits=deg  RzVelocityTargetSpecify=off  RzVelocityTargetPriority=High  RzVelocityTargetValue=0  RzVelocityTargetValueUnits=deg/s
  Check AR angle : checkpacklib/Check Custom Bounds  InstantiateOnLoad=on  enabled=off  stopWhenAssertionFail=off  export=off  ViewDlgPos=[989.8 92 851.2 475.4]  OpenViewOnLoad=off  LaunchViewOnOpen=off  TimeUnits=seconds  EnableUpperBound=on  UpperBoundTimes=[2 3]  UpperBoundAmplitudes=[5 5];  EnableLowerBound=on  LowerBoundTimes=[2 3]  LowerBoundAmplitudes=[-5 -5];
      settings: LibrarySourceBlock=sdolib/Signal Constraints/Check Custom Bounds
  Check FE angle : checkpacklib/Check Custom Bounds  InstantiateOnLoad=on  enabled=off  stopWhenAssertionFail=off  export=off  ViewDlgPos=[287 267 851 475]  OpenViewOnLoad=off  LaunchViewOnOpen=off  TimeUnits=seconds  EnableUpperBound=on  UpperBoundTimes={ [0.7 0.8], [0.2 0.3] }  UpperBoundAmplitudes={ [4.5 4.5], [-3.5 -3.5] }  EnableLowerBound=on  LowerBoundTimes={ [0.7 0.8], [0.2 0.3] }  LowerBoundAmplitudes={ [3.5 3.5], [-4.5 -4.5] }
      settings: LibrarySourceBlock=sdolib/Signal Constraints/Check Custom Bounds
  Check LB angle : checkpacklib/Check Custom Bounds  InstantiateOnLoad=on  enabled=off  stopWhenAssertionFail=off  export=off  ViewDlgPos=[989.8 92 851.2 475.4]  OpenViewOnLoad=off  LaunchViewOnOpen=off  TimeUnits=seconds  EnableUpperBound=on  UpperBoundTimes=[1 2]  UpperBoundAmplitudes=[5 5];  EnableLowerBound=on  LowerBoundTimes=[1 2]  LowerBoundAmplitudes=[-5 -5];
      settings: LibrarySourceBlock=sdolib/Signal Constraints/Check Custom Bounds
  Clock : Clock
  Constant : Constant  Commented=on  Value=30.839
  Constant2 : Constant  Value=14.555
  Constant3 : Constant  Value=0
  Constant4 : Constant  Value=0
  Flexion force at L1 : sm_lib/Forces and Torques/External Force and Torque  ForceResolutionFrame=AttachedFrame  EnableForceX=off  EnableForceY=off  EnableForceZ=off  EnableForce=off  TorqueResolutionFrame=AttachedFrame  EnableTorqueX=on  EnableTorqueY=off  EnableTorqueZ=off  EnableTorque=off
  Gain : Gain  Gain=-1
  Gain1 : Gain  Gain=-1
  Gain2 : Gain  Commented=on  Gain=-1
  Gain3 : Gain  Commented=on  Gain=-1
  IVD4_N : sm_lib/Body Elements/Flexible Bodies/Reduced Order Flexible Solid  GraphicAmbientColor=[0.15 0.15 0.15 1.0]  GraphicDiffuseColor=[0 0.4471 0.7412]  DampingType=Proportional  GraphicEmissiveColor=[0.0 0.0 0.0 1.0]  GraphicFacetVertexIndices=IVD4_N.GraphicFacetVertexIndices  InterfaceFrameOrientations=IVD4_N.InterfaceFrameOrientations  GraphicType=DeformedGeometry  MassMatrix=IVD4_N.MassMatrix  NumRetainedModes=1  NumberOfInterfaceFrames=2  GraphicOpacity=1.0  GraphicReconstructionMatrix=IVD4_N.GraphicReconstructionMatrix  ReductionType=None  InterfaceFrameOrigins=IVD4_N.InterfaceFrameOrigins  GraphicShininess=75  GraphicSpecularColor=[0.5 0.5 0.5 1.0]  StiffnessMatrix=IVD4_N.StiffnessMatrix * E_IVD4_N  GeomUnitType=FromFile  GraphicVertexCoordinates=IVD4_N.GraphicVertexCoordinates  VisRecursionLimit=3  GraphicVisPropType=SimpleVisualProperties  LengthUnit=m  MassUnit=kg  TimeUnit=s  UnitSystemType=SI  ProportionalDampingAlpha=0  ProportionalDampingBeta=0.001  UniformModalDampingRatio=0.01  DampingMatrix=[]
  IVD4_Z1 : sm_lib/Body Elements/Flexible Bodies/Reduced Order Flexible Solid  GraphicAmbientColor=[0.15 0.15 0.15 1.0]  GraphicDiffuseColor=[0.851 0.3255 0.09804]  DampingType=Proportional  GraphicEmissiveColor=[0.0 0.0 0.0 1.0]  GraphicFacetVertexIndices=IVD4_Z1.GraphicFacetVertexIndices  InterfaceFrameOrientations=IVD4_Z1.InterfaceFrameOrientations  GraphicType=DeformedGeometry  MassMatrix=IVD4_Z1.MassMatrix  NumRetainedModes=1  NumberOfInterfaceFrames=2  GraphicOpacity=0.5  GraphicReconstructionMatrix=IVD4_Z1.GraphicReconstructionMatrix  ReductionType=None  InterfaceFrameOrigins=IVD4_Z1.InterfaceFrameOrigins  GraphicShininess=75  GraphicSpecularColor=[0.5 0.5 0.5 1.0]  StiffnessMatrix=IVD4_Z1.StiffnessMatrix * E_IVD4_Z1  GeomUnitType=FromFile  GraphicVertexCoordinates=IVD4_Z1.GraphicVertexCoordinates  VisRecursionLimit=3  GraphicVisPropType=SimpleVisualProperties  LengthUnit=m  MassUnit=kg  TimeUnit=s  UnitSystemType=SI  ProportionalDampingAlpha=0  ProportionalDampingBeta=0.001  UniformModalDampingRatio=0.01  DampingMatrix=[]
  IVD4_Z2 : sm_lib/Body Elements/Flexible Bodies/Reduced Order Flexible Solid  GraphicAmbientColor=[0.15 0.15 0.15 1.0]  GraphicDiffuseColor=[0.9294 0.6941 0.1255]  DampingType=Proportional  GraphicEmissiveColor=[0.0 0.0 0.0 1.0]  GraphicFacetVertexIndices=IVD4_Z2.GraphicFacetVertexIndices  InterfaceFrameOrientations=IVD4_Z2.InterfaceFrameOrientations  GraphicType=DeformedGeometry  MassMatrix=IVD4_Z2.MassMatrix  NumRetainedModes=1  NumberOfInterfaceFrames=2  GraphicOpacity=0.5  GraphicReconstructionMatrix=IVD4_Z2.GraphicReconstructionMatrix  ReductionType=None  InterfaceFrameOrigins=IVD4_Z2.InterfaceFrameOrigins  GraphicShininess=75  GraphicSpecularColor=[0.5 0.5 0.5 1.0]  StiffnessMatrix=IVD4_Z2.StiffnessMatrix * E_IVD4_Z2  GeomUnitType=FromFile  GraphicVertexCoordinates=IVD4_Z2.GraphicVertexCoordinates  VisRecursionLimit=3  GraphicVisPropType=SimpleVisualProperties  LengthUnit=m  MassUnit=kg  TimeUnit=s  UnitSystemType=SI  ProportionalDampingAlpha=0  ProportionalDampingBeta=0.001  UniformModalDampingRatio=0.01  DampingMatrix=[]
  IVD4_Z3 : sm_lib/Body Elements/Flexible Bodies/Reduced Order Flexible Solid  GraphicAmbientColor=[0.15 0.15 0.15 1.0]  GraphicDiffuseColor=[0.4941 0.1843 0.5569]  DampingType=Proportional  GraphicEmissiveColor=[0.0 0.0 0.0 1.0]  GraphicFacetVertexIndices=IVD4_Z3.GraphicFacetVertexIndices  InterfaceFrameOrientations=IVD4_Z3.InterfaceFrameOrientations  GraphicType=DeformedGeometry  MassMatrix=IVD4_Z3.MassMatrix  NumRetainedModes=1  NumberOfInterfaceFrames=2  GraphicOpacity=0.5  GraphicReconstructionMatrix=IVD4_Z3.GraphicReconstructionMatrix  ReductionType=None  InterfaceFrameOrigins=IVD4_Z3.InterfaceFrameOrigins  GraphicShininess=75  GraphicSpecularColor=[0.5 0.5 0.5 1.0]  StiffnessMatrix=IVD4_Z3.StiffnessMatrix * E_IVD4_Z3  GeomUnitType=FromFile  GraphicVertexCoordinates=IVD4_Z3.GraphicVertexCoordinates  VisRecursionLimit=3  GraphicVisPropType=SimpleVisualProperties  LengthUnit=m  MassUnit=kg  TimeUnit=s  UnitSystemType=SI  ProportionalDampingAlpha=0  ProportionalDampingBeta=0.001  UniformModalDampingRatio=0.01  DampingMatrix=[]
  IVD4_Z4 : sm_lib/Body Elements/Flexible Bodies/Reduced Order Flexible Solid  GraphicAmbientColor=[0.15 0.15 0.15 1.0]  GraphicDiffuseColor=[0.4667 0.6745 0.1882]  DampingType=Proportional  GraphicEmissiveColor=[0.0 0.0 0.0 1.0]  GraphicFacetVertexIndices=IVD4_Z4.GraphicFacetVertexIndices  InterfaceFrameOrientations=IVD4_Z4.InterfaceFrameOrientations  GraphicType=DeformedGeometry  MassMatrix=IVD4_Z4.MassMatrix  NumRetainedModes=1  NumberOfInterfaceFrames=2  GraphicOpacity=0.5  GraphicReconstructionMatrix=IVD4_Z4.GraphicReconstructionMatrix  ReductionType=None  InterfaceFrameOrigins=IVD4_Z4.InterfaceFrameOrigins  GraphicShininess=75  GraphicSpecularColor=[0.5 0.5 0.5 1.0]  StiffnessMatrix=IVD4_Z4.StiffnessMatrix * E_IVD4_Z4  GeomUnitType=FromFile  GraphicVertexCoordinates=IVD4_Z4.GraphicVertexCoordinates  VisRecursionLimit=3  GraphicVisPropType=SimpleVisualProperties  LengthUnit=m  MassUnit=kg  TimeUnit=s  UnitSystemType=SI  ProportionalDampingAlpha=0  ProportionalDampingBeta=0.001  UniformModalDampingRatio=0.01  DampingMatrix=[]
  IVD5_N : sm_lib/Body Elements/Flexible Bodies/Reduced Order Flexible Solid  GraphicAmbientColor=[0.15 0.15 0.15 1.0]  GraphicDiffuseColor=[0 0.4471 0.7412]  DampingType=Proportional  GraphicEmissiveColor=[0.0 0.0 0.0 1.0]  GraphicFacetVertexIndices=IVD5_N.GraphicFacetVertexIndices  InterfaceFrameOrientations=IVD5_N.InterfaceFrameOrientations  GraphicType=DeformedGeometry  MassMatrix=IVD5_N.MassMatrix  NumRetainedModes=1  NumberOfInterfaceFrames=2  GraphicOpacity=1.0  GraphicReconstructionMatrix=IVD5_N.GraphicReconstructionMatrix  ReductionType=None  InterfaceFrameOrigins=IVD5_N.InterfaceFrameOrigins  GraphicShininess=75  GraphicSpecularColor=[0.5 0.5 0.5 1.0]  StiffnessMatrix=IVD5_N.StiffnessMatrix * E_IVD5_N  GeomUnitType=FromFile  GraphicVertexCoordinates=IVD5_N.GraphicVertexCoordinates  VisRecursionLimit=3  GraphicVisPropType=SimpleVisualProperties  LengthUnit=m  MassUnit=kg  TimeUnit=s  UnitSystemType=SI  ProportionalDampingAlpha=0  ProportionalDampingBeta=0.001  UniformModalDampingRatio=0.01  DampingMatrix=[]
  IVD5_Z1 : sm_lib/Body Elements/Flexible Bodies/Reduced Order Flexible Solid  GraphicAmbientColor=[0.15 0.15 0.15 1.0]  GraphicDiffuseColor=[0.851 0.3255 0.09804]  DampingType=Proportional  GraphicEmissiveColor=[0.0 0.0 0.0 1.0]  GraphicFacetVertexIndices=IVD5_Z1.GraphicFacetVertexIndices  InterfaceFrameOrientations=IVD5_Z1.InterfaceFrameOrientations  GraphicType=DeformedGeometry  MassMatrix=IVD5_Z1.MassMatrix  NumRetainedModes=1  NumberOfInterfaceFrames=2  GraphicOpacity=0.5  GraphicReconstructionMatrix=IVD5_Z1.GraphicReconstructionMatrix  ReductionType=None  InterfaceFrameOrigins=IVD5_Z1.InterfaceFrameOrigins  GraphicShininess=75  GraphicSpecularColor=[0.5 0.5 0.5 1.0]  StiffnessMatrix=IVD5_Z1.StiffnessMatrix * E_IVD5_Z1  GeomUnitType=FromFile  GraphicVertexCoordinates=IVD5_Z1.GraphicVertexCoordinates  VisRecursionLimit=3  GraphicVisPropType=SimpleVisualProperties  LengthUnit=m  MassUnit=kg  TimeUnit=s  UnitSystemType=SI  ProportionalDampingAlpha=0  ProportionalDampingBeta=0.001  UniformModalDampingRatio=0.01  DampingMatrix=[]
  IVD5_Z2 : sm_lib/Body Elements/Flexible Bodies/Reduced Order Flexible Solid  GraphicAmbientColor=[0.15 0.15 0.15 1.0]  GraphicDiffuseColor=[0.9294 0.6941 0.1255]  DampingType=Proportional  GraphicEmissiveColor=[0.0 0.0 0.0 1.0]  GraphicFacetVertexIndices=IVD5_Z2.GraphicFacetVertexIndices  InterfaceFrameOrientations=IVD5_Z2.InterfaceFrameOrientations  GraphicType=DeformedGeometry  MassMatrix=IVD5_Z2.MassMatrix  NumRetainedModes=1  NumberOfInterfaceFrames=2  GraphicOpacity=0.5  GraphicReconstructionMatrix=IVD5_Z2.GraphicReconstructionMatrix  ReductionType=None  InterfaceFrameOrigins=IVD5_Z2.InterfaceFrameOrigins  GraphicShininess=75  GraphicSpecularColor=[0.5 0.5 0.5 1.0]  StiffnessMatrix=IVD5_Z2.StiffnessMatrix * E_IVD5_Z2  GeomUnitType=FromFile  GraphicVertexCoordinates=IVD5_Z2.GraphicVertexCoordinates  VisRecursionLimit=3  GraphicVisPropType=SimpleVisualProperties  LengthUnit=m  MassUnit=kg  TimeUnit=s  UnitSystemType=SI  ProportionalDampingAlpha=0  ProportionalDampingBeta=0.001  UniformModalDampingRatio=0.01  DampingMatrix=[]
  IVD5_Z3 : sm_lib/Body Elements/Flexible Bodies/Reduced Order Flexible Solid  GraphicAmbientColor=[0.15 0.15 0.15 1.0]  GraphicDiffuseColor=[0.4941 0.1843 0.5569]  DampingType=Proportional  GraphicEmissiveColor=[0.0 0.0 0.0 1.0]  GraphicFacetVertexIndices=IVD5_Z3.GraphicFacetVertexIndices  InterfaceFrameOrientations=IVD5_Z3.InterfaceFrameOrientations  GraphicType=DeformedGeometry  MassMatrix=IVD5_Z3.MassMatrix  NumRetainedModes=1  NumberOfInterfaceFrames=2  GraphicOpacity=0.5  GraphicReconstructionMatrix=IVD5_Z3.GraphicReconstructionMatrix  ReductionType=None  InterfaceFrameOrigins=IVD5_Z3.InterfaceFrameOrigins  GraphicShininess=75  GraphicSpecularColor=[0.5 0.5 0.5 1.0]  StiffnessMatrix=IVD5_Z3.StiffnessMatrix * E_IVD5_Z3  GeomUnitType=FromFile  GraphicVertexCoordinates=IVD5_Z3.GraphicVertexCoordinates  VisRecursionLimit=3  GraphicVisPropType=SimpleVisualProperties  LengthUnit=m  MassUnit=kg  TimeUnit=s  UnitSystemType=SI  ProportionalDampingAlpha=0  ProportionalDampingBeta=0.001  UniformModalDampingRatio=0.01  DampingMatrix=[]
  IVD5_Z4 : sm_lib/Body Elements/Flexible Bodies/Reduced Order Flexible Solid  GraphicAmbientColor=[0.15 0.15 0.15 1.0]  GraphicDiffuseColor=[0.4667 0.6745 0.1882]  DampingType=Proportional  GraphicEmissiveColor=[0.0 0.0 0.0 1.0]  GraphicFacetVertexIndices=IVD5_Z4.GraphicFacetVertexIndices  InterfaceFrameOrientations=IVD5_Z4.InterfaceFrameOrientations  GraphicType=DeformedGeometry  MassMatrix=IVD5_Z4.MassMatrix  NumRetainedModes=1  NumberOfInterfaceFrames=2  GraphicOpacity=0.5  GraphicReconstructionMatrix=IVD5_Z4.GraphicReconstructionMatrix  ReductionType=None  InterfaceFrameOrigins=IVD5_Z4.InterfaceFrameOrigins  GraphicShininess=75  GraphicSpecularColor=[0.5 0.5 0.5 1.0]  StiffnessMatrix=IVD5_Z4.StiffnessMatrix * E_IVD5_Z4  GeomUnitType=FromFile  GraphicVertexCoordinates=IVD5_Z4.GraphicVertexCoordinates  VisRecursionLimit=3  GraphicVisPropType=SimpleVisualProperties  LengthUnit=m  MassUnit=kg  TimeUnit=s  UnitSystemType=SI  ProportionalDampingAlpha=0  ProportionalDampingBeta=0.001  UniformModalDampingRatio=0.01  DampingMatrix=[]
  L4 : sm_lib/Body Elements/File Solid  ExtGeomFileName=C:\Users\siril\OneDrive\Desktop\TIM-Control\Matlab\Simscape models\Reduced Order Model\CAD\model with 5 sections\L4.step  UnitType=FromFile  ExtGeomFileUnits=m  StepReaderType=HEX  ExportConvexHullGeometry=off  InertiaType=CalculateFromGeometry  Mass=1  MassUnits=kg  CenterOfMass=[0 0 0]  CenterOfMassUnits=m  MomentsOfInertia=[1 1 1]  MomentsOfInertiaUnits=kg*m^2  ProductsOfInertia=[0 0 0]  ProductsOfInertiaUnits=kg*m^2  BasedOnType=Density  Density=1  DensityUnits=g/cm^3  DoExposeReferenceFrame=off  SerializedFrames=<Frames><Frame><Id>Frame1</Id><Value><Name>To IVD4_N</Name><Origin><Source>GeometricFeature</Source><FeatureName>planar surface 8</FeatureName></Origin><PrimaryAxis><DefinedDirection>+Z</DefinedDirection><Source>GeometricFeature</Source><SourceDirection>+Z</SourceDirection><FeatureName>planar surface 8</FeatureName></PrimaryAxis><SecondaryAxis><DefinedDirection>+X</DefinedDirection><Source>ReferenceFrame</Source><SourceDirection>+X</SourceDirection><FeatureName></FeatureName></SecondaryAxis></Value></Frame><Frame><Id>Frame2</Id><Value><Name>To IVD4_Z1</Name><Origin><Source>GeometricFeature</Source><FeatureName>planar surface 7</FeatureName></Origin><PrimaryAxis><DefinedDirection>+Z</DefinedDirection><Source>GeometricFeature</Source><SourceDirection>+Z</SourceDirection><FeatureName>planar surface 7</FeatureName></PrimaryAxis><SecondaryAxis><DefinedDirection>+X</DefinedDirection><Source>ReferenceFrame</Source><SourceDirection>+X</SourceDirection><FeatureName></FeatureName></SecondaryAxis></Value></Frame><Frame><Id>Frame3</Id><Value><Name>To IVD4_Z2</Name><Origin><Source>GeometricFeature</Source><FeatureName>planar surface 5</FeatureName></Origin><PrimaryAxis><DefinedDirection>+Z</DefinedDirection><Source>GeometricFeature</Source><SourceDirection>+Z</SourceDirection><FeatureName>planar surface 5</FeatureName></PrimaryAxis><SecondaryAxis><DefinedDirection>+X</DefinedDirection><Source>ReferenceFrame</Source><SourceDirection>+X</SourceDirection><FeatureName></FeatureName></SecondaryAxis></Value></Frame><Frame><Id>Frame4</Id><Value><Name>To IVD4_Z3</Name><Origin><Source>GeometricFeature</Source><FeatureName>planar surface 15</FeatureName></Origin><PrimaryAxis><DefinedDirection>+Z</DefinedDirection><Source>GeometricFeature</Source><SourceDirection>+Z</SourceDirection><FeatureName>planar surface 15</FeatureName></PrimaryAxis><SecondaryAxis><DefinedDirection>+X</DefinedDirection><Source>ReferenceFrame</Source><SourceDirection>+X</SourceDirection><FeatureName></FeatureName></SecondaryAxis></Value></Frame><Frame><Id>Frame5</Id><Value><Name>To IVD4_Z4</Name><Origin><Source>GeometricFeature</Source><FeatureName>planar surface 6</FeatureName></Origin><PrimaryAxis><DefinedDirection>+Z</DefinedDirection><Source>GeometricFeature</Source><SourceDirection>+Z</SourceDirection><FeatureName>planar surface 6</FeatureName></PrimaryAxis><SecondaryAxis><DefinedDirection>+X</DefinedDirection><Source>ReferenceFrame</Source><SourceDirection>+X</SourceDirection><FeatureName></FeatureName></SecondaryAxis></Value></Frame><Frame><Id>Frame6</Id><Value><Name>L4 COM</Name><Origin><Source>CenterOfMassFrame</Source><FeatureName></FeatureName></Origin><PrimaryAxis><DefinedDirection>+Z</DefinedDirection><Source>ReferenceFrame</Source><SourceDirection>+Z</SourceDirection><FeatureName></FeatureName></PrimaryAxis><SecondaryAxis><DefinedDirection>+X</DefinedDirection><Source>ReferenceFrame</Source><SourceDirection>+X</SourceDirection><FeatureName></FeatureName></SecondaryAxis></Value></Frame><Frame><Id>Frame7</Id><Value><Name>To IVD3_N</Name><Origin><Source>GeometricFeature</Source><FeatureName>planar surface 4</FeatureName></Origin><PrimaryAxis><DefinedDirection>-Z</DefinedDirection><Source>GeometricFeature</Source><SourceDirection>+Z</SourceDirection><FeatureName>planar surface 4</FeatureName></PrimaryAxis><SecondaryAxis><DefinedDirection>+X</DefinedDirection><Source>ReferenceFrame</Source><SourceDirection>+X</SourceDirection><FeatureName></FeatureName></SecondaryAxis></Value></Frame><Frame><Id>Frame8</Id><Value><Name>To IVD3_Z1</Name><Origin><Source>GeometricFeature</Source><FeatureName>planar surface 1</FeatureName></Origin><PrimaryAxis><DefinedDirection>-Z</DefinedDirection><Source>GeometricFeature</Source><SourceDirection>+Z</SourceDirection><FeatureName>planar surface 1</FeatureName></PrimaryAxis><SecondaryAxis><DefinedDirection>+X</DefinedDirection><Source>ReferenceFrame</Source><SourceDirection>+X</SourceDirection><FeatureName></FeatureName></SecondaryAxis></Value></Frame><Frame><Id>Frame9</Id><Value><Name>To IVD3_Z2</Name><Origin><Source>GeometricFeature</Source><FeatureName>planar surface 3</FeatureName></Origin><PrimaryAxis><DefinedDirection>-Z</DefinedDirection><Source>GeometricFeature</Source><SourceDirection>+Z</SourceDirection><FeatureName>planar surface 3</FeatureName></PrimaryAxis><SecondaryAxis><DefinedDirection>+X</DefinedDirection><Source>ReferenceFrame</Source><SourceDirection>+X</SourceDirection><FeatureName></FeatureName></SecondaryAxis></Value></Frame><Frame><Id>Frame10</Id><Value><Name>To IVD3_Z3</Name><Origin><Source>GeometricFeature</Source><FeatureName>planar surface 2</FeatureName></Origin><PrimaryAxis><DefinedDirection>-Z</DefinedDirection><Source>GeometricFeature</Source><SourceDirection>+Z</SourceDirection><FeatureName>planar surface 2</FeatureName></PrimaryAxis><SecondaryAxis><DefinedDirection>+X</DefinedDirection><Source>ReferenceFrame</Source><SourceDirection>+X</SourceDirection><FeatureName></FeatureName></SecondaryAxis></Value></Frame><Frame><Id>Frame11</Id><Value><Name>To IVD3_Z4</Name><Origin><Source>GeometricFeature</Source><FeatureName>planar surface 72</FeatureName></Origin><PrimaryAxis><DefinedDirection>-Z</DefinedDirection><Source>GeometricFeature</Source><SourceDirection>+Z</SourceDirection><FeatureName>planar surface 72</FeatureName></PrimaryAxis><SecondaryAxis><DefinedDirection>+X</DefinedDirection><Source>ReferenceFrame</Source><SourceDirection>+X</SourceDirection><FeatureName></FeatureName></SecondaryAxis></Value></Frame></Frames>  GraphicType=FromGeometry  MarkerShape=Sphere  MarkerSize=10  GraphicVisPropType=SimpleVisualProperties  GraphicDiffuseColor=[0.5 0.5 0.5]  GraphicSpecularColor=[0.5 0.5 0.5 1.0]  GraphicAmbientColor=[0.15 0.15 0.15 1.0]  GraphicEmissiveColor=[0.0 0.0 0.0 1.0]  GraphicShininess=75  GraphicOpacity=1.0
  L5 : sm_lib/Body Elements/File Solid  ExtGeomFileName=C:\Users\siril\OneDrive\Desktop\TIM-Control\Matlab\Simscape models\Reduced Order Model\CAD\model with 5 sections\L5.step  UnitType=FromFile  ExtGeomFileUnits=m  StepReaderType=HEX  ExportConvexHullGeometry=off  InertiaType=CalculateFromGeometry  Mass=1  MassUnits=kg  CenterOfMass=[0 0 0]  CenterOfMassUnits=m  MomentsOfInertia=[1 1 1]  MomentsOfInertiaUnits=kg*m^2  ProductsOfInertia=[0 0 0]  ProductsOfInertiaUnits=kg*m^2  BasedOnType=Density  Density=0.18  DensityUnits=g/cm^3  DoExposeReferenceFrame=off  SerializedFrames=<Frames><Frame><Id>Frame1</Id><Value><Name>To IVD5_N</Name><Origin><Source>GeometricFeature</Source><FeatureName>planar surface 8</FeatureName></Origin><PrimaryAxis><DefinedDirection>+Z</DefinedDirection><Source>GeometricFeature</Source><SourceDirection>+Z</SourceDirection><FeatureName>planar surface 8</FeatureName></PrimaryAxis><SecondaryAxis><DefinedDirection>+X</DefinedDirection><Source>ReferenceFrame</Source><SourceDirection>+X</SourceDirection><FeatureName></FeatureName></SecondaryAxis></Value></Frame><Frame><Id>Frame2</Id><Value><Name>To IVD5_Z1</Name><Origin><Source>GeometricFeature</Source><FeatureName>planar surface 7</FeatureName></Origin><PrimaryAxis><DefinedDirection>+Z</DefinedDirection><Source>GeometricFeature</Source><SourceDirection>+Z</SourceDirection><FeatureName>planar surface 7</FeatureName></PrimaryAxis><SecondaryAxis><DefinedDirection>+X</DefinedDirection><Source>ReferenceFrame</Source><SourceDirection>+X</SourceDirection><FeatureName></FeatureName></SecondaryAxis></Value></Frame><Frame><Id>Frame3</Id><Value><Name>To IVD5_Z2</Name><Origin><Source>GeometricFeature</Source><FeatureName>planar surface 6</FeatureName></Origin><PrimaryAxis><DefinedDirection>+Z</DefinedDirection><Source>GeometricFeature</Source><SourceDirection>+Z</SourceDirection><FeatureName>planar surface 6</FeatureName></PrimaryAxis><SecondaryAxis><DefinedDirection>+X</DefinedDirection><Source>ReferenceFrame</Source><SourceDirection>+X</SourceDirection><FeatureName></FeatureName></SecondaryAxis></Value></Frame><Frame><Id>Frame4</Id><Value><Name>To IVD5_Z3</Name><Origin><Source>GeometricFeature</Source><FeatureName>planar surface 2767</FeatureName></Origin><PrimaryAxis><DefinedDirection>+Z</DefinedDirection><Source>GeometricFeature</Source><SourceDirection>+Z</SourceDirection><FeatureName>planar surface 2767</FeatureName></PrimaryAxis><SecondaryAxis><DefinedDirection>+X</DefinedDirection><Source>ReferenceFrame</Source><SourceDirection>+X</SourceDirection><FeatureName></FeatureName></SecondaryAxis></Value></Frame><Frame><Id>Frame5</Id><Value><Name>To IVD5_Z4</Name><Origin><Source>GeometricFeature</Source><FeatureName>planar surface 5</FeatureName></Origin><PrimaryAxis><DefinedDirection>+Z</DefinedDirection><Source>GeometricFeature</Source><SourceDirection>+Z</SourceDirection><FeatureName>planar surface 5</FeatureName></PrimaryAxis><SecondaryAxis><DefinedDirection>+X</DefinedDirection><Source>ReferenceFrame</Source><SourceDirection>+X</SourceDirection><FeatureName></FeatureName></SecondaryAxis></Value></Frame><Frame><Id>Frame6</Id><Value><Name>L5 COM</Name><Origin><Source>CenterOfMassFrame</Source><FeatureName></FeatureName></Origin><PrimaryAxis><DefinedDirection>+Z</DefinedDirection><Source>ReferenceFrame</Source><SourceDirection>+Z</SourceDirection><FeatureName></FeatureName></PrimaryAxis><SecondaryAxis><DefinedDirection>+X</DefinedDirection><Source>ReferenceFrame</Source><SourceDirection>+X</SourceDirection><FeatureName></FeatureName></SecondaryAxis></Value></Frame><Frame><Id>Frame7</Id><Value><Name>To IVD4_N</Name><Origin><Source>GeometricFeature</Source><FeatureName>planar surface 4</FeatureName></Origin><PrimaryAxis><DefinedDirection>-Z</DefinedDirection><Source>GeometricFeature</Source><SourceDirection>+Z</SourceDirection><FeatureName>planar surface 4</FeatureName></PrimaryAxis><SecondaryAxis><DefinedDirection>+X</DefinedDirection><Source>ReferenceFrame</Source><SourceDirection>+X</SourceDirection><FeatureName></FeatureName></SecondaryAxis></Value></Frame><Frame><Id>Frame8</Id><Value><Name>To IVD4_Z1</Name><Origin><Source>GeometricFeature</Source><FeatureName>planar surface 3</FeatureName></Origin><PrimaryAxis><DefinedDirection>-Z</DefinedDirection><Source>GeometricFeature</Source><SourceDirection>+Z</SourceDirection><FeatureName>planar surface 3</FeatureName></PrimaryAxis><SecondaryAxis><DefinedDirection>+X</DefinedDirection><Source>ReferenceFrame</Source><SourceDirection>+X</SourceDirection><FeatureName></FeatureName></SecondaryAxis></Value></Frame><Frame><Id>Frame9</Id><Value><Name>To IVD4_Z2</Name><Origin><Source>GeometricFeature</Source><FeatureName>planar surface 1</FeatureName></Origin><PrimaryAxis><DefinedDirection>-Z</DefinedDirection><Source>GeometricFeature</Source><SourceDirection>+Z</SourceDirection><FeatureName>planar surface 1</FeatureName></PrimaryAxis><SecondaryAxis><DefinedDirection>+X</DefinedDirection><Source>ReferenceFrame</Source><SourceDirection>+X</SourceDirection><FeatureName></FeatureName></SecondaryAxis></Value></Frame><Frame><Id>Frame10</Id><Value><Name>To IVD4_Z3</Name><Origin><Source>GeometricFeature</Source><FeatureName>planar surface 2705</FeatureName></Origin><PrimaryAxis><DefinedDirection>-Z</DefinedDirection><Source>GeometricFeature</Source><SourceDirection>+Z</SourceDirection><FeatureName>planar surface 2705</FeatureName></PrimaryAxis><SecondaryAxis><DefinedDirection>+X</DefinedDirection><Source>ReferenceFrame</Source><SourceDirection>+X</SourceDirection><FeatureName></FeatureName></SecondaryAxis></Value></Frame><Frame><Id>Frame11</Id><Value><Name>To IVD4_Z4</Name><Origin><Source>GeometricFeature</Source><FeatureName>planar surface 2</FeatureName></Origin><PrimaryAxis><DefinedDirection>-Z</DefinedDirection><Source>GeometricFeature</Source><SourceDirection>+Z</SourceDirection><FeatureName>planar surface 2</FeatureName></PrimaryAxis><SecondaryAxis><DefinedDirection>+X</DefinedDirection><Source>ReferenceFrame</Source><SourceDirection>+X</SourceDirection><FeatureName></FeatureName></SecondaryAxis></Value></Frame></Frames>  GraphicType=FromGeometry  MarkerShape=Sphere  MarkerSize=10  GraphicVisPropType=SimpleVisualProperties  GraphicDiffuseColor=[0.5 0.5 0.5]  GraphicSpecularColor=[0.5 0.5 0.5 1.0]  GraphicAmbientColor=[0.15 0.15 0.15 1.0]  GraphicEmissiveColor=[0.0 0.0 0.0 1.0]  GraphicShininess=75  GraphicOpacity=1.0
  L5-S1 Flexion : checkpacklib/Check Against Reference  Commented=on  InstantiateOnLoad=on  enabled=off  stopWhenAssertionFail=off  export=off  ViewDlgPos=[1127.4 348.2 509.6 389.6]  OpenViewOnLoad=off  LaunchViewOnOpen=off  TimeUnits=seconds  EnableReferenceBound=on  AbsTolerance=eps^(1/3)  RelTolerance=0.01  ReferenceTimes=|  ReferenceAmplitudes=|
      ReferenceTimes=|
      | [0
      | 0.14052587
      | 0.279158534
      | 0.424951626
      | 0.571147428
      | 0.706826793
      | 0.856093048
      | 1]
      ReferenceAmplitudes=|
      | [0
      | 1.496288519
      | 2.573872723
      | 3.533527255
      | 4.390295876
      | 5.022609363
      | 5.697018069
      | 6.278868701]
      settings: LibrarySourceBlock=sdolib/Signal Constraints/Check Against Reference
  MATLAB Function : MATLAB Function  TreatAsAtomicUnit=on
  Mechanism Configuration : sm_lib/Utilities/Mechanism Configuration  UniformGravity=Constant  GravityVector=[0 0 -9.80665]  GravityVectorUnits=m/s^2  LinearizationDelta=0.001  JointModeTransitionNonlinearIterations=2
  Moment_AR : Sin  Amplitude=Moment_AR  Frequency=7  SampleTime=0
  Moment_FE : Sin  Amplitude=-Moment_FE  Frequency=7  SampleTime=0
  Moment_LB : Sin  Amplitude=-Moment_LB  Frequency=7  SampleTime=0
  PS-Simulink Converter : nesl_utility/PS-Simulink Converter  Commented=on  PhysicalDomain=network_engine_domain  SubClassName=ps_output  LeftPortType=input  RightPortType=output  PseudoPeriodic=off  Frequencies=[]  VectorFormat=inherit  Unit=inherit  AffineConversion=off
  PS-Simulink Converter1 : nesl_utility/PS-Simulink Converter  PhysicalDomain=network_engine_domain  SubClassName=ps_output  LeftPortType=input  RightPortType=output  PseudoPeriodic=off  Frequencies=[]  VectorFormat=inherit  Unit=inherit  AffineConversion=off
  PS-Simulink Converter5 : nesl_utility/PS-Simulink Converter  PhysicalDomain=network_engine_domain  SubClassName=ps_output  LeftPortType=input  RightPortType=output  PseudoPeriodic=off  Frequencies=[]  VectorFormat=inherit  Unit=inherit  AffineConversion=off
  PS-Simulink Converter9 : nesl_utility/PS-Simulink Converter  PhysicalDomain=network_engine_domain  SubClassName=ps_output  LeftPortType=input  RightPortType=output  PseudoPeriodic=off  Frequencies=[]  VectorFormat=inherit  Unit=inherit  AffineConversion=off
  Pure AR Moment at L1 COM : sm_lib/Forces and Torques/External Force and Torque  ForceResolutionFrame=World  EnableForceX=off  EnableForceY=off  EnableForceZ=off  EnableForce=off  TorqueResolutionFrame=World  EnableTorqueX=off  EnableTorqueY=off  EnableTorqueZ=on  EnableTorque=off
  Pure FE Moment at L1 COM : sm_lib/Forces and Torques/External Force and Torque  ForceResolutionFrame=World  EnableForceX=off  EnableForceY=off  EnableForceZ=off  EnableForce=off  TorqueResolutionFrame=World  EnableTorqueX=on  EnableTorqueY=off  EnableTorqueZ=off  EnableTorque=off
  Pure LB Moment at L1 COM : sm_lib/Forces and Torques/External Force and Torque  ForceResolutionFrame=World  EnableForceX=off  EnableForceY=off  EnableForceZ=off  EnableForce=off  TorqueResolutionFrame=World  EnableTorqueX=off  EnableTorqueY=on  EnableTorqueZ=off  EnableTorque=off
  Radians to Degrees : simulink_extras/Transformations/Radians to Degrees  Commented=on
  Radians to Degrees1 : simulink_extras/Transformations/Radians to Degrees
  Radians to Degrees2 : simulink_extras/Transformations/Radians to Degrees
  Radians to Degrees4 : simulink_extras/Transformations/Radians to Degrees
  Ramp : simulink/Sources/Ramp  slope=0  start=0  InitialOutput=0
  S1 : sm_lib/Body Elements/File Solid  ExtGeomFileName=C:\Users\siril\OneDrive\Desktop\TIM-Control\Matlab\Simscape models\Reduced Order Model\CAD\model with 5 sections\S1.step  UnitType=FromFile  ExtGeomFileUnits=m  StepReaderType=HEX  ExportConvexHullGeometry=off  InertiaType=CalculateFromGeometry  Mass=1  MassUnits=kg  CenterOfMass=[0 0 0]  CenterOfMassUnits=m  MomentsOfInertia=[1 1 1]  MomentsOfInertiaUnits=kg*m^2  ProductsOfInertia=[0 0 0]  ProductsOfInertiaUnits=kg*m^2  BasedOnType=Density  Density=1  DensityUnits=g/cm^3  DoExposeReferenceFrame=on  SerializedFrames=<Frames><Frame><Id>Frame1</Id><Value><Name>To IVD5_N</Name><Origin><Source>GeometricFeature</Source><FeatureName>planar surface 4</FeatureName></Origin><PrimaryAxis><DefinedDirection>+Z</DefinedDirection><Source>GeometricFeature</Source><SourceDirection>+Z</SourceDirection><FeatureName>planar surface 4</FeatureName></PrimaryAxis><SecondaryAxis><DefinedDirection>+X</DefinedDirection><Source>ReferenceFrame</Source><SourceDirection>+X</SourceDirection><FeatureName></FeatureName></SecondaryAxis></Value></Frame><Frame><Id>Frame2</Id><Value><Name>To IVD5_Z1</Name><Origin><Source>GeometricFeature</Source><FeatureName>planar surface 1</FeatureName></Origin><PrimaryAxis><DefinedDirection>+Z</DefinedDirection><Source>GeometricFeature</Source><SourceDirection>+Z</SourceDirection><FeatureName>planar surface 1</FeatureName></PrimaryAxis><SecondaryAxis><DefinedDirection>+X</DefinedDirection><Source>ReferenceFrame</Source><SourceDirection>+X</SourceDirection><FeatureName></FeatureName></SecondaryAxis></Value></Frame><Frame><Id>Frame3</Id><Value><Name>To IVD5_Z2</Name><Origin><Source>GeometricFeature</Source><FeatureName>planar surface 3</FeatureName></Origin><PrimaryAxis><DefinedDirection>+Z</DefinedDirection><Source>GeometricFeature</Source><SourceDirection>+Z</SourceDirection><FeatureName>planar surface 3</FeatureName></PrimaryAxis><SecondaryAxis><DefinedDirection>+X</DefinedDirection><Source>ReferenceFrame</Source><SourceDirection>+X</SourceDirection><FeatureName></FeatureName></SecondaryAxis></Value></Frame><Frame><Id>Frame4</Id><Value><Name>To IVD5_Z3</Name><Origin><Source>GeometricFeature</Source><FeatureName>planar surface 12326</FeatureName></Origin><PrimaryAxis><DefinedDirection>+Z</DefinedDirection><Source>GeometricFeature</Source><SourceDirection>+Z</SourceDirection><FeatureName>planar surface 12326</FeatureName></PrimaryAxis><SecondaryAxis><DefinedDirection>+X</DefinedDirection><Source>ReferenceFrame</Source><SourceDirection>+X</SourceDirection><FeatureName></FeatureName></SecondaryAxis></Value></Frame><Frame><Id>Frame5</Id><Value><Name>To IVD5_Z4</Name><Origin><Source>GeometricFeature</Source><FeatureName>planar surface 2</FeatureName></Origin><PrimaryAxis><DefinedDirection>+Z</DefinedDirection><Source>GeometricFeature</Source><SourceDirection>+Z</SourceDirection><FeatureName>planar surface 2</FeatureName></PrimaryAxis><SecondaryAxis><DefinedDirection>+X</DefinedDirection><Source>ReferenceFrame</Source><SourceDirection>+X</SourceDirection><FeatureName></FeatureName></SecondaryAxis></Value></Frame></Frames>  GraphicType=FromGeometry  MarkerShape=Sphere  MarkerSize=10  GraphicVisPropType=SimpleVisualProperties  GraphicDiffuseColor=[0.5 0.5 0.5]  GraphicSpecularColor=[0.5 0.5 0.5 1.0]  GraphicAmbientColor=[0.15 0.15 0.15 1.0]  GraphicEmissiveColor=[0.0 0.0 0.0 1.0]  GraphicShininess=75  GraphicOpacity=1.0
  Scope : Scope
  Scope1 : Scope  NumInputPorts=3
  Scope2 : Scope  Commented=on
  Scope3 : Scope  NumInputPorts=3
  Simulink-PS Converter{1..4} (4 alike) : nesl_utility/Simulink-PS Converter  PhysicalDomain=network_engine_domain  SubClassName=ps_input  LeftPortType=input  RightPortType=output  PseudoPeriodic=off  Frequencies=[]  NoiseDistribution=none  NoiseParameters=[]  Unit=1  AffineConversion=off  FilteringAndDerivatives=provide  SimscapeFilterOrder=1  InputFilterTimeConstant=0.001  UdotUserProvided=0
  Solver Configuration : nesl_utility/Solver Configuration  PhysicalDomain=network_engine_domain  SubClassName=solver  LeftPortType=input  RightPortType=generic  Tones=[]  Harmonics=[]  SimulateNoise=off  Profile=off  UseLocalSampling=off  EnableSwitchedLinearOptims=on  FrequencyDomain=off  UseCCode=off  RelTol=0.001  AbsTol=1e-06  MinStep=1e-09  ToWorkspace=off  RevertToSquareIcSolve=off  NumHomotopyIterations=100  PhasorMode=off  PhasorModeNumHarmonics=1  ConsistencySolver=NEWTON_FTOL  IndexReductionMethod=DerivativeReplacement  DoDC=off  ResidualTolerance=1e-04  ConsistencyTolSource=GLOBAL  ConsistencyAbsTol=0.001  ConsistencyRelTol=0.001  ConsistencyTolFactor=0.001  UseLocalSolver=off  LocalSolverChoice=NE_BACKWARD_EULER_ADVANCER  ResolveIndetEquations=on  FunctionEvalNumThread=1  LocalSolverSampleTime=0.001  DoFixedCost=off  MaxNonlinIter=3  MaxModeIter=2  ComputeImpulses=off  ImpulseIterations=2  LinearAlgebra=Sparse  LinearAlgebraNumThread=0  EquationFormulation=NE_TIME_EF  DelaysMemoryBudget=1024  AutomaticFiltering=on  FilteringTimeConstant=0.001  PartitionStorageMethod=AS_NEEDED  PartitionMemoryBudget=1024  PartitionMethod=FAST
  Weld Joint{,1..7} (8 alike) : sm_lib/Joints/Weld Joint  JointMode=Normal  SenseConstraintForce=off  SenseConstraintForceX=off  SenseConstraintForceY=off  SenseConstraintForceZ=off  SenseConstraintTorque=off  SenseConstraintTorqueX=off  SenseConstraintTorqueY=off  SenseConstraintTorqueZ=off  SenseTotalForce=off  SenseTotalForceX=off  SenseTotalForceY=off  SenseTotalForceZ=off  SenseTotalTorque=off  SenseTotalTorqueX=off  SenseTotalTorqueY=off  SenseTotalTorqueZ=off  CompositeWrenchDir=FollowerOnBase  CompositeWrenchFrame=BaseFrame
  World Frame : sm_lib/Frames and Transforms/World Frame
  XY Graph : Record  Commented=on  FileSettingsInternal="{\"entries\":[{\"content\":{\"excelSettings\":{\"content\":{},\"type\":\"Streamout.ExcelSettings\"}},\"type\":\"Streamout.FileSettingStorage\",\"uuid\":\"db32a2b6-01b3-4cb2-8e04-05ca1e0c382c\"}],\"packageUris\":[\"http://schema.mathworks.com/mf0/streamout_blocks/R2020a\"],\"version\":\"1.0\"}"  Layout=[1 1]  SignalsInternal="{\"entries\":[{\"content\":{},\"type\":\"RecordBlkView.InputSignals\",\"uuid\":\"ecb6f1a4-8602-45a6-a5ea-bb03adc8715f\"}],\"packageUris\":[\"http://schema.mathworks.com/mf0/streamout_blocks/R2020a\"],\"version\":\"1.0\"}"  VisualizationBindings="{\"xyplotplugin\":{\"info\":[{\"series\":[],\"subplotID\":1}]}}"  CompatibilityTag=XY
  wires:
  Radians to Degrees2/1 -> Add2/1
  PS-Simulink Converter1/1 -> Radians to Degrees1/1
  Radians to Degrees4/1 -> Add/1, Scope/1
  PS-Simulink Converter5/1 -> Radians to Degrees2/1
  Radians to Degrees1/1 -> Add1/1
  Constant4/1 -> Add2/2
  Constant3/1 -> Add/2, Add1/2
  Add1/1 -> Gain1/1
  Add/1 -> Gain/1
  Gain/1 -> Check FE angle/1, Scope1/1  "FE"
  Gain1/1 -> Check LB angle/1, Scope1/2  "LB"
  Add2/1 -> Check AR angle/1, Scope1/3  "AR"
  Moment_FE/1 -> Gain3/1
  Ramp/1 -> Simulink-PS Converter1/1
  PS-Simulink Converter9/1 -> Radians to Degrees4/1
  PS-Simulink Converter/1 -> Radians to Degrees/1
  Radians to Degrees/1 -> Add3/1
  Add3/1 -> Gain2/1
  Constant/1 -> Add3/2
  Gain2/1 -> L5-S1 Flexion/1, XY Graph/2, Scope2/1  "L5-S1 FE Rot"
  Gain3/1 -> XY Graph/1  "L5-S1 FE Rot"
  MATLAB Function/1(FE) -> Simulink-PS Converter2/1, Scope3/1  "FEmoment"
  Clock/1 -> MATLAB Function/1(t)
  MATLAB Function/2(LB) -> Scope3/2, Simulink-PS Converter3/1  "LBmoment"
  MATLAB Function/3(AR) -> Simulink-PS Converter4/1, Scope3/3  "ARmoment"
  connections:
  World Frame/RConn1 -- Mechanism Configuration/RConn1 -- Bushing Joint/LConn1 -- S1/RConn1 -- Solver Configuration/RConn1
  Bushing Joint/RConn2 -- PS-Simulink Converter9/LConn1
  Bushing Joint/RConn3 -- PS-Simulink Converter1/LConn1
  Bushing Joint/RConn4 -- PS-Simulink Converter5/LConn1
  Flexion force at L1/RConn1 -- L4/RConn3 -- Bushing Joint/RConn1 -- Pure AR Moment at L1 COM/RConn1 -- Pure LB Moment at L1 COM/RConn1 -- Pure FE Moment at L1 COM/RConn1
  Simulink-PS Converter1/RConn1 -- Flexion force at L1/LConn1
  Pure LB Moment at L1 COM/LConn1 -- Simulink-PS Converter3/RConn1
  Simulink-PS Converter2/RConn1 -- Pure FE Moment at L1 COM/LConn1
  Simulink-PS Converter4/RConn1 -- Pure AR Moment at L1 COM/LConn1
  PS-Simulink Converter/LConn1 -- Bushing Joint1/RConn2
  IVD5_N/LConn1 -- S1/LConn1
  L5/LConn1 -- IVD5_N/RConn1
  IVD5_Z1/LConn1 -- S1/LConn2
  Weld Joint/LConn1 -- IVD5_Z1/RConn1
  Weld Joint/RConn1 -- L5/RConn1
  IVD5_Z2/LConn1 -- S1/RConn2
  Weld Joint1/LConn1 -- IVD5_Z2/RConn1
  Weld Joint1/RConn1 -- L5/LConn2
  IVD5_Z3/LConn1 -- S1/LConn3
  IVD5_Z3/RConn1 -- Weld Joint2/LConn1
  Weld Joint2/RConn1 -- L5/RConn2
  IVD5_Z4/LConn1 -- S1/RConn3
  Weld Joint3/LConn1 -- IVD5_Z4/RConn1
  Weld Joint3/RConn1 -- L5/LConn3
  IVD4_N/LConn1 -- L5/LConn4
  IVD4_N/RConn1 -- L4/LConn1
  IVD4_Z1/LConn1 -- L5/RConn4
  IVD4_Z1/RConn1 -- Weld Joint4/LConn1
  Weld Joint4/RConn1 -- L4/RConn1
  IVD4_Z2/LConn1 -- L5/LConn5
  IVD4_Z2/RConn1 -- Weld Joint5/LConn1
  Weld Joint5/RConn1 -- L4/LConn2
  IVD4_Z3/RConn1 -- Weld Joint6/LConn1
  IVD4_Z3/LConn1 -- L5/RConn5
  Weld Joint6/RConn1 -- L4/RConn2
  IVD4_Z4/LConn1 -- L5/LConn6
  IVD4_Z4/RConn1 -- Weld Joint7/LConn1
  Weld Joint7/RConn1 -- L4/LConn3
